simulink model "Model2"  (R2017a)
settings: Solver=ode23t  StartTime=0.0  StopTime=10.0  RelTol=1e-4
values from neighbouring files (symbols this model uses):
  param = evalin('base','param')    [getSaveInfo.m]    (also in loadBackUp.m)
(part 2 of 3)

== matlab function Model2/PodwojnyIntegrator/ObiektOdsprzegniety/Dynamika ==
  data: u input; zp output; q input; qp input; z input
function zp = fcn(u,q,qp,z)

c1=cos(q(6));
c3=cos(q(8));

s1=sin(q(6));
s3=sin(q(8));

invQ=[(0.679340444444444444E4+(-0.384000000000000000E3).*c1.^2+ ...
  0.407936888888888889E4.*c3+0.512000000000000000E3.*c1.*c3+( ...
  -0.170666666666666667E3).*c1.^2.*c3+(-0.162203728395061728E4).* ...
  c3.^2+0.113777777777777778E3.*c1.*c3.^2+0.125037037037037037E3.* ...
  c1.^2.*c3.^2+(-0.145391148148148148E4).*c3.^3+( ...
  -0.192000000000000000E3).*c1.*c3.^3+0.640000000000000000E2.* ...
  c1.^2.*c3.^3+(-0.347058518518518519E3).*c3.^4+( ...
  -0.426666666666666667E2).*c1.*c3.^4+0.711111111111111111E1.* ...
  c1.^2.*c3.^4+(-0.284444444444444444E2).*c3.^5+( ...
  -0.115200000000000000E4).*c1.*s1+0.768000000000000000E3.*c3.*s1+( ...
  -0.512000000000000000E3).*c1.*c3.*s1+0.170666666666666667E3.* ...
  c3.^2.*s1+0.375111111111111111E3.*c1.*c3.^2.*s1+( ...
  -0.288000000000000000E3).*c3.^3.*s1+0.192000000000000000E3.*c1.* ...
  c3.^3.*s1+(-0.640000000000000000E2).*c3.^4.*s1+ ...
  0.213333333333333333E2.*c1.*c3.^4.*s1+(-0.864000000000000000E3).* ...
  s1.^2+(-0.384000000000000000E3).*c3.*s1.^2+ ...
  0.281333333333333333E3.*c3.^2.*s1.^2+0.144000000000000000E3.* ...
  c3.^3.*s1.^2+0.160000000000000000E2.*c3.^4.*s1.^2+( ...
  -0.384000000000000000E3).*c1.^2.*s3.^2+(-0.192000000000000000E3).* ...
  c1.^2.*c3.*s3.^2+(-0.426666666666666667E2).*c1.^2.*c3.^2.*s3.^2+ ...
  0.512000000000000000E3.*c1.*s1.*s3.^2+0.256000000000000000E3.*c1.* ...
  c3.*s1.*s3.^2+0.568888888888888889E2.*c1.*c3.^2.*s1.*s3.^2+( ...
  -0.170666666666666667E3).*s1.^2.*s3.^2+(-0.853333333333333333E2).* ...
  c3.*s1.^2.*s3.^2+(-0.189629629629629630E2).*c3.^2.*s1.^2.*s3.^2).* ...
  (0.175621873777777778E7+0.E-37.*c1+(-0.236544000000000000E6).* ...
  c1.^2+0.129863203555555556E7.*c3+0.315392000000000000E6.*c1.*c3+( ...
  -0.105130666666666667E6).*c1.^2.*c3+(-0.358315944691358025E6).* ...
  c3.^2+0.700871111111111111E5.*c1.*c3.^2+0.770228148148148148E5.* ...
  c1.^2.*c3.^2+(-0.440262272592592593E6).*c3.^3+( ...
  -0.118272000000000000E6).*c1.*c3.^3+0.394240000000000000E5.* ...
  c1.^2.*c3.^3+(-0.112599780740740741E6).*c3.^4+( ...
  -0.262826666666666667E5).*c1.*c3.^4+0.438044444444444444E4.* ...
  c1.^2.*c3.^4+(-0.175217777777777778E5).*c3.^5+0.E-39.*c1.*c3.^5+ ...
  0.E-39.*c3.^6+0.E-36.*s1+0.E-37.*c1.*s1+0.E-37.*c3.*s1+0.E-37.* ...
  c1.*c3.*s1+0.E-37.*c3.^2.*s1+0.E-37.*c1.*c3.^2.*s1+0.E-37.*c3.^3.* ...
  s1+0.E-38.*c1.*c3.^3.*s1+0.E-38.*c3.^4.*s1+0.E-39.*c1.*c3.^4.*s1+ ...
  0.E-39.*c3.^5.*s1+(-0.384885600000000000E6).*s1.^2+( ...
  -0.263220266666666667E6).*c3.*s1.^2+0.843654037037037037E5.* ...
  c3.^2.*s1.^2+0.941564888888888889E5.*c3.^3.*s1.^2+ ...
  0.224875111111111111E5.*c3.^4.*s1.^2+0.170666666666666667E4.* ...
  c3.^5.*s1.^2+(-0.171060266666666667E6).*c1.^2.*s3.^2+ ...
  0.230400000000000000E5.*c1.^4.*s3.^2+(-0.126490133333333333E6).* ...
  c1.^2.*c3.*s3.^2+(-0.307200000000000000E5).*c1.^3.*c3.*s3.^2+ ...
  0.102400000000000000E5.*c1.^4.*c3.*s3.^2+(-0.292466962962962963E5) ...
  .*c1.^2.*c3.^2.*s3.^2+(-0.682666666666666667E4).*c1.^3.*c3.^2.* ...
  s3.^2+0.113777777777777778E4.*c1.^4.*c3.^2.*s3.^2+( ...
  -0.455111111111111111E4).*c1.^2.*c3.^3.*s3.^2+0.E-37.*c1.*s1.* ...
  s3.^2+0.E-37.*c1.*c3.*s1.*s3.^2+0.E-38.*c1.*c3.^2.*s1.*s3.^2+( ...
  -0.105130666666666667E6).*s1.^2.*s3.^2+0.460800000000000000E5.* ...
  c1.^2.*s1.^2.*s3.^2+(-0.525653333333333333E5).*c3.*s1.^2.*s3.^2+( ...
  -0.307200000000000000E5).*c1.*c3.*s1.^2.*s3.^2+ ...
  0.204800000000000000E5.*c1.^2.*c3.*s1.^2.*s3.^2+( ...
  -0.116811851851851852E5).*c3.^2.*s1.^2.*s3.^2+( ...
  -0.682666666666666667E4).*c1.*c3.^2.*s1.^2.*s3.^2+ ...
  0.227555555555555556E4.*c1.^2.*c3.^2.*s1.^2.*s3.^2+ ...
  0.230400000000000000E5.*s1.^4.*s3.^2+0.102400000000000000E5.*c3.* ...
  s1.^4.*s3.^2+0.113777777777777778E4.*c3.^2.*s1.^4.*s3.^2).^(-1),(( ...
  -0.109139555555555556E4)+(-0.384000000000000000E3).*c1.^2+ ...
  0.136968888888888889E3.*c3+0.512000000000000000E3.*c1.*c3+( ...
  -0.170666666666666667E3).*c1.^2.*c3+0.458673827160493827E3.*c3.^2+ ...
  0.113777777777777778E3.*c1.*c3.^2+0.125037037037037037E3.*c1.^2.* ...
  c3.^2+0.244885185185185185E2.*c3.^3+(-0.192000000000000000E3).* ...
  c1.*c3.^3+0.640000000000000000E2.*c1.^2.*c3.^3+( ...
  -0.185251851851851852E2).*c3.^4+(-0.426666666666666667E2).*c1.* ...
  c3.^4+0.711111111111111111E1.*c1.^2.*c3.^4+( ...
  -0.284444444444444444E2).*c3.^5+0.864000000000000000E3.*s1.^2+ ...
  0.384000000000000000E3.*c3.*s1.^2+(-0.281333333333333333E3).* ...
  c3.^2.*s1.^2+(-0.144000000000000000E3).*c3.^3.*s1.^2+( ...
  -0.160000000000000000E2).*c3.^4.*s1.^2+0.384000000000000000E3.* ...
  c1.^2.*s3.^2+0.192000000000000000E3.*c1.^2.*c3.*s3.^2+ ...
  0.426666666666666667E2.*c1.^2.*c3.^2.*s3.^2+( ...
  -0.170666666666666667E3).*s1.^2.*s3.^2+(-0.853333333333333333E2).* ...
  c3.*s1.^2.*s3.^2+(-0.189629629629629630E2).*c3.^2.*s1.^2.*s3.^2).* ...
  (0.175621873777777778E7+0.E-37.*c1+(-0.236544000000000000E6).* ...
  c1.^2+0.129863203555555556E7.*c3+0.315392000000000000E6.*c1.*c3+( ...
  -0.105130666666666667E6).*c1.^2.*c3+(-0.358315944691358025E6).* ...
  c3.^2+0.700871111111111111E5.*c1.*c3.^2+0.770228148148148148E5.* ...
  c1.^2.*c3.^2+(-0.440262272592592593E6).*c3.^3+( ...
  -0.118272000000000000E6).*c1.*c3.^3+0.394240000000000000E5.* ...
  c1.^2.*c3.^3+(-0.112599780740740741E6).*c3.^4+( ...
  -0.262826666666666667E5).*c1.*c3.^4+0.438044444444444444E4.* ...
  c1.^2.*c3.^4+(-0.175217777777777778E5).*c3.^5+0.E-39.*c1.*c3.^5+ ...
  0.E-39.*c3.^6+0.E-36.*s1+0.E-37.*c1.*s1+0.E-37.*c3.*s1+0.E-37.* ...
  c1.*c3.*s1+0.E-37.*c3.^2.*s1+0.E-37.*c1.*c3.^2.*s1+0.E-37.*c3.^3.* ...
  s1+0.E-38.*c1.*c3.^3.*s1+0.E-38.*c3.^4.*s1+0.E-39.*c1.*c3.^4.*s1+ ...
  0.E-39.*c3.^5.*s1+(-0.384885600000000000E6).*s1.^2+( ...
  -0.263220266666666667E6).*c3.*s1.^2+0.843654037037037037E5.* ...
  c3.^2.*s1.^2+0.941564888888888889E5.*c3.^3.*s1.^2+ ...
  0.224875111111111111E5.*c3.^4.*s1.^2+0.170666666666666667E4.* ...
  c3.^5.*s1.^2+(-0.171060266666666667E6).*c1.^2.*s3.^2+ ...
  0.230400000000000000E5.*c1.^4.*s3.^2+(-0.126490133333333333E6).* ...
  c1.^2.*c3.*s3.^2+(-0.307200000000000000E5).*c1.^3.*c3.*s3.^2+ ...
  0.102400000000000000E5.*c1.^4.*c3.*s3.^2+(-0.292466962962962963E5) ...
  .*c1.^2.*c3.^2.*s3.^2+(-0.682666666666666667E4).*c1.^3.*c3.^2.* ...
  s3.^2+0.113777777777777778E4.*c1.^4.*c3.^2.*s3.^2+( ...
  -0.455111111111111111E4).*c1.^2.*c3.^3.*s3.^2+0.E-37.*c1.*s1.* ...
  s3.^2+0.E-37.*c1.*c3.*s1.*s3.^2+0.E-38.*c1.*c3.^2.*s1.*s3.^2+( ...
  -0.105130666666666667E6).*s1.^2.*s3.^2+0.460800000000000000E5.* ...
  c1.^2.*s1.^2.*s3.^2+(-0.525653333333333333E5).*c3.*s1.^2.*s3.^2+( ...
  -0.307200000000000000E5).*c1.*c3.*s1.^2.*s3.^2+ ...
  0.204800000000000000E5.*c1.^2.*c3.*s1.^2.*s3.^2+( ...
  -0.116811851851851852E5).*c3.^2.*s1.^2.*s3.^2+( ...
  -0.682666666666666667E4).*c1.*c3.^2.*s1.^2.*s3.^2+ ...
  0.227555555555555556E4.*c1.^2.*c3.^2.*s1.^2.*s3.^2+ ...
  0.230400000000000000E5.*s1.^4.*s3.^2+0.102400000000000000E5.*c3.* ...
  s1.^4.*s3.^2+0.113777777777777778E4.*c3.^2.*s1.^4.*s3.^2).^(-1),(( ...
  -0.262826666666666667E5)+(-0.197120000000000000E5).*c1+( ...
  -0.438044444444444444E4).*c1.*c3+0.693570370370370370E4.*c3.^2+ ...
  0.739200000000000000E4.*c1.*c3.^2+0.164266666666666667E4.*c1.* ...
  c3.^3+0.109511111111111111E4.*c3.^4+0.213825333333333333E5.*s1+ ...
  0.384000000000000000E4.*c1.*s1+0.731167407407407407E4.*c3.*s1+ ...
  0.170666666666666667E4.*c1.*c3.*s1+(-0.744956111111111111E4).* ...
  c3.^2.*s1+(-0.125037037037037037E4).*c1.*c3.^2.*s1+( ...
  -0.274187777777777778E4).*c3.^3.*s1+(-0.640000000000000000E3).* ...
  c1.*c3.^3.*s1+(-0.213333333333333333E3).*c3.^4.*s1+( ...
  -0.711111111111111111E2).*c1.*c3.^4.*s1+0.576000000000000000E4.* ...
  s1.^2+0.256000000000000000E4.*c3.*s1.^2+(-0.187555555555555556E4) ...
  .*c3.^2.*s1.^2+(-0.960000000000000000E3).*c3.^3.*s1.^2+( ...
  -0.106666666666666667E3).*c3.^4.*s1.^2+0.256000000000000000E4.* ...
  c1.^2.*s3.^2+0.192000000000000000E4.*c1.^3.*s3.^2+ ...
  0.426666666666666667E3.*c1.^3.*c3.*s3.^2+0.284444444444444444E3.* ...
  c1.^2.*c3.^2.*s3.^2+(-0.170666666666666667E4).*c1.*s1.*s3.^2+( ...
  -0.128000000000000000E4).*c1.^2.*s1.*s3.^2+( ...
  -0.284444444444444444E3).*c1.^2.*c3.*s1.*s3.^2+( ...
  -0.189629629629629630E3).*c1.*c3.^2.*s1.*s3.^2+ ...
  0.192000000000000000E4.*c1.*s1.^2.*s3.^2+0.426666666666666667E3.* ...
  c1.*c3.*s1.^2.*s3.^2+(-0.128000000000000000E4).*s1.^3.*s3.^2+( ...
  -0.284444444444444444E3).*c3.*s1.^3.*s3.^2).*( ...
  0.175621873777777778E7+0.E-37.*c1+(-0.236544000000000000E6).* ...
  c1.^2+0.129863203555555556E7.*c3+0.315392000000000000E6.*c1.*c3+( ...
  -0.105130666666666667E6).*c1.^2.*c3+(-0.358315944691358025E6).* ...
  c3.^2+0.700871111111111111E5.*c1.*c3.^2+0.770228148148148148E5.* ...
  c1.^2.*c3.^2+(-0.440262272592592593E6).*c3.^3+( ...
  -0.118272000000000000E6).*c1.*c3.^3+0.394240000000000000E5.* ...
  c1.^2.*c3.^3+(-0.112599780740740741E6).*c3.^4+( ...
  -0.262826666666666667E5).*c1.*c3.^4+0.438044444444444444E4.* ...
  c1.^2.*c3.^4+(-0.175217777777777778E5).*c3.^5+0.E-39.*c1.*c3.^5+ ...
  0.E-39.*c3.^6+0.E-36.*s1+0.E-37.*c1.*s1+0.E-37.*c3.*s1+0.E-37.* ...
  c1.*c3.*s1+0.E-37.*c3.^2.*s1+0.E-37.*c1.*c3.^2.*s1+0.E-37.*c3.^3.* ...
  s1+0.E-38.*c1.*c3.^3.*s1+0.E-38.*c3.^4.*s1+0.E-39.*c1.*c3.^4.*s1+ ...
  0.E-39.*c3.^5.*s1+(-0.384885600000000000E6).*s1.^2+( ...
  -0.263220266666666667E6).*c3.*s1.^2+0.843654037037037037E5.* ...
  c3.^2.*s1.^2+0.941564888888888889E5.*c3.^3.*s1.^2+ ...
  0.224875111111111111E5.*c3.^4.*s1.^2+0.170666666666666667E4.* ...
  c3.^5.*s1.^2+(-0.171060266666666667E6).*c1.^2.*s3.^2+ ...
  0.230400000000000000E5.*c1.^4.*s3.^2+(-0.126490133333333333E6).* ...
  c1.^2.*c3.*s3.^2+(-0.307200000000000000E5).*c1.^3.*c3.*s3.^2+ ...
  0.102400000000000000E5.*c1.^4.*c3.*s3.^2+(-0.292466962962962963E5) ...
  .*c1.^2.*c3.^2.*s3.^2+(-0.682666666666666667E4).*c1.^3.*c3.^2.* ...
  s3.^2+0.113777777777777778E4.*c1.^4.*c3.^2.*s3.^2+( ...
  -0.455111111111111111E4).*c1.^2.*c3.^3.*s3.^2+0.E-37.*c1.*s1.* ...
  s3.^2+0.E-37.*c1.*c3.*s1.*s3.^2+0.E-38.*c1.*c3.^2.*s1.*s3.^2+( ...
  -0.105130666666666667E6).*s1.^2.*s3.^2+0.460800000000000000E5.* ...
  c1.^2.*s1.^2.*s3.^2+(-0.525653333333333333E5).*c3.*s1.^2.*s3.^2+( ...
  -0.307200000000000000E5).*c1.*c3.*s1.^2.*s3.^2+ ...
  0.204800000000000000E5.*c1.^2.*c3.*s1.^2.*s3.^2+( ...
  -0.116811851851851852E5).*c3.^2.*s1.^2.*s3.^2+( ...
  -0.682666666666666667E4).*c1.*c3.^2.*s1.^2.*s3.^2+ ...
  0.227555555555555556E4.*c1.^2.*c3.^2.*s1.^2.*s3.^2+ ...
  0.230400000000000000E5.*s1.^4.*s3.^2+0.102400000000000000E5.*c3.* ...
  s1.^4.*s3.^2+0.113777777777777778E4.*c3.^2.*s1.^4.*s3.^2).^(-1),(( ...
  -0.213825333333333333E4).*c1.*c3.*s3+0.288000000000000000E3.* ...
  c1.^3.*c3.*s3+(-0.158112666666666667E4).*c1.*c3.^2.*s3+( ...
  -0.384000000000000000E3).*c1.^2.*c3.^2.*s3+ ...
  0.128000000000000000E3.*c1.^3.*c3.^2.*s3+(-0.365583703703703704E3) ...
  .*c1.*c3.^3.*s3+(-0.853333333333333333E2).*c1.^2.*c3.^3.*s3+ ...
  0.142222222222222222E2.*c1.^3.*c3.^3.*s3+(-0.568888888888888889E2) ...
  .*c1.*c3.^4.*s3+(-0.197120000000000000E4).*c3.*s1.*s3+ ...
  0.432000000000000000E3.*c1.^2.*c3.*s1.*s3+( ...
  -0.985600000000000000E3).*c3.^2.*s1.*s3+(-0.288000000000000000E3) ...
  .*c1.*c3.^2.*s1.*s3+0.192000000000000000E3.*c1.^2.*c3.^2.*s1.*s3+( ...
  -0.219022222222222222E3).*c3.^3.*s1.*s3+(-0.640000000000000000E2) ...
  .*c1.*c3.^3.*s1.*s3+0.213333333333333333E2.*c1.^2.*c3.^3.*s1.*s3+ ...
  0.288000000000000000E3.*c1.*c3.*s1.^2.*s3+( ...
  -0.192000000000000000E3).*c3.^2.*s1.^2.*s3+ ...
  0.128000000000000000E3.*c1.*c3.^2.*s1.^2.*s3+( ...
  -0.426666666666666667E2).*c3.^3.*s1.^2.*s3+ ...
  0.142222222222222222E2.*c1.*c3.^3.*s1.^2.*s3+ ...
  0.432000000000000000E3.*c3.*s1.^3.*s3+0.192000000000000000E3.* ...
  c3.^2.*s1.^3.*s3+0.213333333333333333E2.*c3.^3.*s1.^3.*s3).*( ...
  0.175621873777777778E7+0.E-37.*c1+(-0.236544000000000000E6).* ...
  c1.^2+0.129863203555555556E7.*c3+0.315392000000000000E6.*c1.*c3+( ...
  -0.105130666666666667E6).*c1.^2.*c3+(-0.358315944691358025E6).* ...
  c3.^2+0.700871111111111111E5.*c1.*c3.^2+0.770228148148148148E5.* ...
  c1.^2.*c3.^2+(-0.440262272592592593E6).*c3.^3+( ...
  -0.118272000000000000E6).*c1.*c3.^3+0.394240000000000000E5.* ...
  c1.^2.*c3.^3+(-0.112599780740740741E6).*c3.^4+( ...
  -0.262826666666666667E5).*c1.*c3.^4+0.438044444444444444E4.* ...
  c1.^2.*c3.^4+(-0.175217777777777778E5).*c3.^5+0.E-39.*c1.*c3.^5+ ...
  0.E-39.*c3.^6+0.E-36.*s1+0.E-37.*c1.*s1+0.E-37.*c3.*s1+0.E-37.* ...
  c1.*c3.*s1+0.E-37.*c3.^2.*s1+0.E-37.*c1.*c3.^2.*s1+0.E-37.*c3.^3.* ...
  s1+0.E-38.*c1.*c3.^3.*s1+0.E-38.*c3.^4.*s1+0.E-39.*c1.*c3.^4.*s1+ ...
  0.E-39.*c3.^5.*s1+(-0.384885600000000000E6).*s1.^2+( ...
  -0.263220266666666667E6).*c3.*s1.^2+0.843654037037037037E5.* ...
  c3.^2.*s1.^2+0.941564888888888889E5.*c3.^3.*s1.^2+ ...
  0.224875111111111111E5.*c3.^4.*s1.^2+0.170666666666666667E4.* ...
  c3.^5.*s1.^2+(-0.171060266666666667E6).*c1.^2.*s3.^2+ ...
  0.230400000000000000E5.*c1.^4.*s3.^2+(-0.126490133333333333E6).* ...
  c1.^2.*c3.*s3.^2+(-0.307200000000000000E5).*c1.^3.*c3.*s3.^2+ ...
  0.102400000000000000E5.*c1.^4.*c3.*s3.^2+(-0.292466962962962963E5) ...
  .*c1.^2.*c3.^2.*s3.^2+(-0.682666666666666667E4).*c1.^3.*c3.^2.* ...
  s3.^2+0.113777777777777778E4.*c1.^4.*c3.^2.*s3.^2+( ...
  -0.455111111111111111E4).*c1.^2.*c3.^3.*s3.^2+0.E-37.*c1.*s1.* ...
  s3.^2+0.E-37.*c1.*c3.*s1.*s3.^2+0.E-38.*c1.*c3.^2.*s1.*s3.^2+( ...
  -0.105130666666666667E6).*s1.^2.*s3.^2+0.460800000000000000E5.* ...
  c1.^2.*s1.^2.*s3.^2+(-0.525653333333333333E5).*c3.*s1.^2.*s3.^2+( ...
  -0.307200000000000000E5).*c1.*c3.*s1.^2.*s3.^2+ ...
  0.204800000000000000E5.*c1.^2.*c3.*s1.^2.*s3.^2+( ...
  -0.116811851851851852E5).*c3.^2.*s1.^2.*s3.^2+( ...
  -0.682666666666666667E4).*c1.*c3.^2.*s1.^2.*s3.^2+ ...
  0.227555555555555556E4.*c1.^2.*c3.^2.*s1.^2.*s3.^2+ ...
  0.230400000000000000E5.*s1.^4.*s3.^2+0.102400000000000000E5.*c3.* ...
  s1.^4.*s3.^2+0.113777777777777778E4.*c3.^2.*s1.^4.*s3.^2).^(-1),( ...
  0.427650666666666667E5.*c1.*s3+(-0.576000000000000000E4).*c1.^3.* ...
  s3+0.316225333333333333E5.*c1.*c3.*s3+0.768000000000000000E4.* ...
  c1.^2.*c3.*s3+(-0.256000000000000000E4).*c1.^3.*c3.*s3+ ...
  0.731167407407407407E4.*c1.*c3.^2.*s3+0.170666666666666667E4.* ...
  c1.^2.*c3.^2.*s3+(-0.284444444444444444E3).*c1.^3.*c3.^2.*s3+ ...
  0.113777777777777778E4.*c1.*c3.^3.*s3+0.394240000000000000E5.*s1.* ...
  s3+(-0.864000000000000000E4).*c1.^2.*s1.*s3+ ...
  0.197120000000000000E5.*c3.*s1.*s3+0.576000000000000000E4.*c1.* ...
  c3.*s1.*s3+(-0.384000000000000000E4).*c1.^2.*c3.*s1.*s3+ ...
  0.438044444444444444E4.*c3.^2.*s1.*s3+0.128000000000000000E4.*c1.* ...
  c3.^2.*s1.*s3+(-0.426666666666666667E3).*c1.^2.*c3.^2.*s1.*s3+( ...
  -0.576000000000000000E4).*c1.*s1.^2.*s3+0.384000000000000000E4.* ...
  c3.*s1.^2.*s3+(-0.256000000000000000E4).*c1.*c3.*s1.^2.*s3+ ...
  0.853333333333333333E3.*c3.^2.*s1.^2.*s3+(-0.284444444444444444E3) ...
  .*c1.*c3.^2.*s1.^2.*s3+(-0.864000000000000000E4).*s1.^3.*s3+( ...
  -0.384000000000000000E4).*c3.*s1.^3.*s3+(-0.426666666666666667E3) ...
  .*c3.^2.*s1.^3.*s3).*(0.175621873777777778E7+0.E-37.*c1+( ...
  -0.236544000000000000E6).*c1.^2+0.129863203555555556E7.*c3+ ...
  0.315392000000000000E6.*c1.*c3+(-0.105130666666666667E6).*c1.^2.* ...
  c3+(-0.358315944691358025E6).*c3.^2+0.700871111111111111E5.*c1.* ...
  c3.^2+0.770228148148148148E5.*c1.^2.*c3.^2+( ...
  -0.440262272592592593E6).*c3.^3+(-0.118272000000000000E6).*c1.* ...
  c3.^3+0.394240000000000000E5.*c1.^2.*c3.^3+( ...
  -0.112599780740740741E6).*c3.^4+(-0.262826666666666667E5).*c1.* ...
  c3.^4+0.438044444444444444E4.*c1.^2.*c3.^4+( ...
  -0.175217777777777778E5).*c3.^5+0.E-39.*c1.*c3.^5+0.E-39.*c3.^6+ ...
  0.E-36.*s1+0.E-37.*c1.*s1+0.E-37.*c3.*s1+0.E-37.*c1.*c3.*s1+ ...
  0.E-37.*c3.^2.*s1+0.E-37.*c1.*c3.^2.*s1+0.E-37.*c3.^3.*s1+0.E-38.* ...
  c1.*c3.^3.*s1+0.E-38.*c3.^4.*s1+0.E-39.*c1.*c3.^4.*s1+0.E-39.* ...
  c3.^5.*s1+(-0.384885600000000000E6).*s1.^2+( ...
  -0.263220266666666667E6).*c3.*s1.^2+0.843654037037037037E5.* ...
  c3.^2.*s1.^2+0.941564888888888889E5.*c3.^3.*s1.^2+ ...
  0.224875111111111111E5.*c3.^4.*s1.^2+0.170666666666666667E4.* ...
  c3.^5.*s1.^2+(-0.171060266666666667E6).*c1.^2.*s3.^2+ ...
  0.230400000000000000E5.*c1.^4.*s3.^2+(-0.126490133333333333E6).* ...
  c1.^2.*c3.*s3.^2+(-0.307200000000000000E5).*c1.^3.*c3.*s3.^2+ ...
  0.102400000000000000E5.*c1.^4.*c3.*s3.^2+(-0.292466962962962963E5) ...
  .*c1.^2.*c3.^2.*s3.^2+(-0.682666666666666667E4).*c1.^3.*c3.^2.* ...
  s3.^2+0.113777777777777778E4.*c1.^4.*c3.^2.*s3.^2+( ...
  -0.455111111111111111E4).*c1.^2.*c3.^3.*s3.^2+0.E-37.*c1.*s1.* ...
  s3.^2+0.E-37.*c1.*c3.*s1.*s3.^2+0.E-38.*c1.*c3.^2.*s1.*s3.^2+( ...
  -0.105130666666666667E6).*s1.^2.*s3.^2+0.460800000000000000E5.* ...
  c1.^2.*s1.^2.*s3.^2+(-0.525653333333333333E5).*c3.*s1.^2.*s3.^2+( ...
  -0.307200000000000000E5).*c1.*c3.*s1.^2.*s3.^2+ ...
  0.204800000000000000E5.*c1.^2.*c3.*s1.^2.*s3.^2+( ...
  -0.116811851851851852E5).*c3.^2.*s1.^2.*s3.^2+( ...
  -0.682666666666666667E4).*c1.*c3.^2.*s1.^2.*s3.^2+ ...
  0.227555555555555556E4.*c1.^2.*c3.^2.*s1.^2.*s3.^2+ ...
  0.230400000000000000E5.*s1.^4.*s3.^2+0.102400000000000000E5.*c3.* ...
  s1.^4.*s3.^2+0.113777777777777778E4.*c3.^2.*s1.^4.*s3.^2).^(-1);(( ...
  -0.109139555555555556E4)+(-0.384000000000000000E3).*c1.^2+ ...
  0.136968888888888889E3.*c3+0.512000000000000000E3.*c1.*c3+( ...
  -0.170666666666666667E3).*c1.^2.*c3+0.458673827160493827E3.*c3.^2+ ...
  0.113777777777777778E3.*c1.*c3.^2+0.125037037037037037E3.*c1.^2.* ...
  c3.^2+0.244885185185185185E2.*c3.^3+(-0.192000000000000000E3).* ...
  c1.*c3.^3+0.640000000000000000E2.*c1.^2.*c3.^3+( ...
  -0.185251851851851852E2).*c3.^4+(-0.426666666666666667E2).*c1.* ...
  c3.^4+0.711111111111111111E1.*c1.^2.*c3.^4+( ...
  -0.284444444444444444E2).*c3.^5+0.864000000000000000E3.*s1.^2+ ...
  0.384000000000000000E3.*c3.*s1.^2+(-0.281333333333333333E3).* ...
  c3.^2.*s1.^2+(-0.144000000000000000E3).*c3.^3.*s1.^2+( ...
  -0.160000000000000000E2).*c3.^4.*s1.^2+0.384000000000000000E3.* ...
  c1.^2.*s3.^2+0.192000000000000000E3.*c1.^2.*c3.*s3.^2+ ...
  0.426666666666666667E2.*c1.^2.*c3.^2.*s3.^2+( ...
  -0.170666666666666667E3).*s1.^2.*s3.^2+(-0.853333333333333333E2).* ...
  c3.*s1.^2.*s3.^2+(-0.189629629629629630E2).*c3.^2.*s1.^2.*s3.^2).* ...
  (0.175621873777777778E7+0.E-37.*c1+(-0.236544000000000000E6).* ...
  c1.^2+0.129863203555555556E7.*c3+0.315392000000000000E6.*c1.*c3+( ...
  -0.105130666666666667E6).*c1.^2.*c3+(-0.358315944691358025E6).* ...
  c3.^2+0.700871111111111111E5.*c1.*c3.^2+0.770228148148148148E5.* ...
  c1.^2.*c3.^2+(-0.440262272592592593E6).*c3.^3+( ...
  -0.118272000000000000E6).*c1.*c3.^3+0.394240000000000000E5.* ...
  c1.^2.*c3.^3+(-0.112599780740740741E6).*c3.^4+( ...
  -0.262826666666666667E5).*c1.*c3.^4+0.438044444444444444E4.* ...
  c1.^2.*c3.^4+(-0.175217777777777778E5).*c3.^5+0.E-39.*c1.*c3.^5+ ...
  0.E-39.*c3.^6+0.E-36.*s1+0.E-37.*c1.*s1+0.E-37.*c3.*s1+0.E-37.* ...
  c1.*c3.*s1+0.E-37.*c3.^2.*s1+0.E-37.*c1.*c3.^2.*s1+0.E-37.*c3.^3.* ...
  s1+0.E-38.*c1.*c3.^3.*s1+0.E-38.*c3.^4.*s1+0.E-39.*c1.*c3.^4.*s1+ ...
  0.E-39.*c3.^5.*s1+(-0.384885600000000000E6).*s1.^2+( ...
  -0.263220266666666667E6).*c3.*s1.^2+0.843654037037037037E5.* ...
  c3.^2.*s1.^2+0.941564888888888889E5.*c3.^3.*s1.^2+ ...
  0.224875111111111111E5.*c3.^4.*s1.^2+0.170666666666666667E4.* ...
  c3.^5.*s1.^2+(-0.171060266666666667E6).*c1.^2.*s3.^2+ ...
  0.230400000000000000E5.*c1.^4.*s3.^2+(-0.126490133333333333E6).* ...
  c1.^2.*c3.*s3.^2+(-0.307200000000000000E5).*c1.^3.*c3.*s3.^2+ ...
  0.102400000000000000E5.*c1.^4.*c3.*s3.^2+(-0.292466962962962963E5) ...
  .*c1.^2.*c3.^2.*s3.^2+(-0.682666666666666667E4).*c1.^3.*c3.^2.* ...
  s3.^2+0.113777777777777778E4.*c1.^4.*c3.^2.*s3.^2+( ...
  -0.455111111111111111E4).*c1.^2.*c3.^3.*s3.^2+0.E-37.*c1.*s1.* ...
  s3.^2+0.E-37.*c1.*c3.*s1.*s3.^2+0.E-38.*c1.*c3.^2.*s1.*s3.^2+( ...
  -0.105130666666666667E6).*s1.^2.*s3.^2+0.460800000000000000E5.* ...
  c1.^2.*s1.^2.*s3.^2+(-0.525653333333333333E5).*c3.*s1.^2.*s3.^2+( ...
  -0.307200000000000000E5).*c1.*c3.*s1.^2.*s3.^2+ ...
  0.204800000000000000E5.*c1.^2.*c3.*s1.^2.*s3.^2+( ...
  -0.116811851851851852E5).*c3.^2.*s1.^2.*s3.^2+( ...
  -0.682666666666666667E4).*c1.*c3.^2.*s1.^2.*s3.^2+ ...
  0.227555555555555556E4.*c1.^2.*c3.^2.*s1.^2.*s3.^2+ ...
  0.230400000000000000E5.*s1.^4.*s3.^2+0.102400000000000000E5.*c3.* ...
  s1.^4.*s3.^2+0.113777777777777778E4.*c3.^2.*s1.^4.*s3.^2).^(-1),( ...
  0.679340444444444444E4+(-0.384000000000000000E3).*c1.^2+ ...
  0.407936888888888889E4.*c3+0.512000000000000000E3.*c1.*c3+( ...
  -0.170666666666666667E3).*c1.^2.*c3+(-0.162203728395061728E4).* ...
  c3.^2+0.113777777777777778E3.*c1.*c3.^2+0.125037037037037037E3.* ...
  c1.^2.*c3.^2+(-0.145391148148148148E4).*c3.^3+( ...
  -0.192000000000000000E3).*c1.*c3.^3+0.640000000000000000E2.* ...
  c1.^2.*c3.^3+(-0.347058518518518519E3).*c3.^4+( ...
  -0.426666666666666667E2).*c1.*c3.^4+0.711111111111111111E1.* ...
  c1.^2.*c3.^4+(-0.284444444444444444E2).*c3.^5+ ...
  0.115200000000000000E4.*c1.*s1+(-0.768000000000000000E3).*c3.*s1+ ...
  0.512000000000000000E3.*c1.*c3.*s1+(-0.170666666666666667E3).* ...
  c3.^2.*s1+(-0.375111111111111111E3).*c1.*c3.^2.*s1+ ...
  0.288000000000000000E3.*c3.^3.*s1+(-0.192000000000000000E3).*c1.* ...
  c3.^3.*s1+0.640000000000000000E2.*c3.^4.*s1+( ...
  -0.213333333333333333E2).*c1.*c3.^4.*s1+(-0.864000000000000000E3) ...
  .*s1.^2+(-0.384000000000000000E3).*c3.*s1.^2+ ...
  0.281333333333333333E3.*c3.^2.*s1.^2+0.144000000000000000E3.* ...
  c3.^3.*s1.^2+0.160000000000000000E2.*c3.^4.*s1.^2+( ...
  -0.384000000000000000E3).*c1.^2.*s3.^2+(-0.192000000000000000E3).* ...
  c1.^2.*c3.*s3.^2+(-0.426666666666666667E2).*c1.^2.*c3.^2.*s3.^2+( ...
  -0.512000000000000000E3).*c1.*s1.*s3.^2+(-0.256000000000000000E3) ...
  .*c1.*c3.*s1.*s3.^2+(-0.568888888888888889E2).*c1.*c3.^2.*s1.* ...
  s3.^2+(-0.170666666666666667E3).*s1.^2.*s3.^2+( ...
  -0.853333333333333333E2).*c3.*s1.^2.*s3.^2+( ...
  -0.189629629629629630E2).*c3.^2.*s1.^2.*s3.^2).*( ...
  0.175621873777777778E7+0.E-37.*c1+(-0.236544000000000000E6).* ...
  c1.^2+0.129863203555555556E7.*c3+0.315392000000000000E6.*c1.*c3+( ...
  -0.105130666666666667E6).*c1.^2.*c3+(-0.358315944691358025E6).* ...
  c3.^2+0.700871111111111111E5.*c1.*c3.^2+0.770228148148148148E5.* ...
  c1.^2.*c3.^2+(-0.440262272592592593E6).*c3.^3+( ...
  -0.118272000000000000E6).*c1.*c3.^3+0.394240000000000000E5.* ...
  c1.^2.*c3.^3+(-0.112599780740740741E6).*c3.^4+( ...
  -0.262826666666666667E5).*c1.*c3.^4+0.438044444444444444E4.* ...
  c1.^2.*c3.^4+(-0.175217777777777778E5).*c3.^5+0.E-39.*c1.*c3.^5+ ...
  0.E-39.*c3.^6+0.E-36.*s1+0.E-37.*c1.*s1+0.E-37.*c3.*s1+0.E-37.* ...
  c1.*c3.*s1+0.E-37.*c3.^2.*s1+0.E-37.*c1.*c3.^2.*s1+0.E-37.*c3.^3.* ...
  s1+0.E-38.*c1.*c3.^3.*s1+0.E-38.*c3.^4.*s1+0.E-39.*c1.*c3.^4.*s1+ ...
  0.E-39.*c3.^5.*s1+(-0.384885600000000000E6).*s1.^2+( ...
  -0.263220266666666667E6).*c3.*s1.^2+0.843654037037037037E5.* ...
  c3.^2.*s1.^2+0.941564888888888889E5.*c3.^3.*s1.^2+ ...
  0.224875111111111111E5.*c3.^4.*s1.^2+0.170666666666666667E4.* ...
  c3.^5.*s1.^2+(-0.171060266666666667E6).*c1.^2.*s3.^2+ ...
  0.230400000000000000E5.*c1.^4.*s3.^2+(-0.126490133333333333E6).* ...
  c1.^2.*c3.*s3.^2+(-0.307200000000000000E5).*c1.^3.*c3.*s3.^2+ ...
  0.102400000000000000E5.*c1.^4.*c3.*s3.^2+(-0.292466962962962963E5) ...
  .*c1.^2.*c3.^2.*s3.^2+(-0.682666666666666667E4).*c1.^3.*c3.^2.* ...
  s3.^2+0.113777777777777778E4.*c1.^4.*c3.^2.*s3.^2+( ...
  -0.455111111111111111E4).*c1.^2.*c3.^3.*s3.^2+0.E-37.*c1.*s1.* ...
  s3.^2+0.E-37.*c1.*c3.*s1.*s3.^2+0.E-38.*c1.*c3.^2.*s1.*s3.^2+( ...
  -0.105130666666666667E6).*s1.^2.*s3.^2+0.460800000000000000E5.* ...
  c1.^2.*s1.^2.*s3.^2+(-0.525653333333333333E5).*c3.*s1.^2.*s3.^2+( ...
  -0.307200000000000000E5).*c1.*c3.*s1.^2.*s3.^2+ ...
  0.204800000000000000E5.*c1.^2.*c3.*s1.^2.*s3.^2+( ...
  -0.116811851851851852E5).*c3.^2.*s1.^2.*s3.^2+( ...
  -0.682666666666666667E4).*c1.*c3.^2.*s1.^2.*s3.^2+ ...
  0.227555555555555556E4.*c1.^2.*c3.^2.*s1.^2.*s3.^2+ ...
  0.230400000000000000E5.*s1.^4.*s3.^2+0.102400000000000000E5.*c3.* ...
  s1.^4.*s3.^2+0.113777777777777778E4.*c3.^2.*s1.^4.*s3.^2).^(-1),( ...
  0.262826666666666667E5+0.197120000000000000E5.*c1+ ...
  0.438044444444444444E4.*c1.*c3+(-0.693570370370370370E4).*c3.^2+( ...
  -0.739200000000000000E4).*c1.*c3.^2+(-0.164266666666666667E4).* ...
  c1.*c3.^3+(-0.109511111111111111E4).*c3.^4+ ...
  0.213825333333333333E5.*s1+0.384000000000000000E4.*c1.*s1+ ...
  0.731167407407407407E4.*c3.*s1+0.170666666666666667E4.*c1.*c3.*s1+ ...
  (-0.744956111111111111E4).*c3.^2.*s1+(-0.125037037037037037E4).* ...
  c1.*c3.^2.*s1+(-0.274187777777777778E4).*c3.^3.*s1+( ...
  -0.640000000000000000E3).*c1.*c3.^3.*s1+(-0.213333333333333333E3) ...
  .*c3.^4.*s1+(-0.711111111111111111E2).*c1.*c3.^4.*s1+( ...
  -0.576000000000000000E4).*s1.^2+(-0.256000000000000000E4).*c3.* ...
  s1.^2+0.187555555555555556E4.*c3.^2.*s1.^2+ ...
  0.960000000000000000E3.*c3.^3.*s1.^2+0.106666666666666667E3.* ...
  c3.^4.*s1.^2+(-0.256000000000000000E4).*c1.^2.*s3.^2+( ...
  -0.192000000000000000E4).*c1.^3.*s3.^2+(-0.426666666666666667E3).* ...
  c1.^3.*c3.*s3.^2+(-0.284444444444444444E3).*c1.^2.*c3.^2.*s3.^2+( ...
  -0.170666666666666667E4).*c1.*s1.*s3.^2+(-0.128000000000000000E4) ...
  .*c1.^2.*s1.*s3.^2+(-0.284444444444444444E3).*c1.^2.*c3.*s1.* ...
  s3.^2+(-0.189629629629629630E3).*c1.*c3.^2.*s1.*s3.^2+( ...
  -0.192000000000000000E4).*c1.*s1.^2.*s3.^2+( ...
  -0.426666666666666667E3).*c1.*c3.*s1.^2.*s3.^2+( ...
  -0.128000000000000000E4).*s1.^3.*s3.^2+(-0.284444444444444444E3).* ...
  c3.*s1.^3.*s3.^2).*(0.175621873777777778E7+0.E-37.*c1+( ...
  -0.236544000000000000E6).*c1.^2+0.129863203555555556E7.*c3+ ...
  0.315392000000000000E6.*c1.*c3+(-0.105130666666666667E6).*c1.^2.* ...
  c3+(-0.358315944691358025E6).*c3.^2+0.700871111111111111E5.*c1.* ...
  c3.^2+0.770228148148148148E5.*c1.^2.*c3.^2+( ...
  -0.440262272592592593E6).*c3.^3+(-0.118272000000000000E6).*c1.* ...
  c3.^3+0.394240000000000000E5.*c1.^2.*c3.^3+( ...
  -0.112599780740740741E6).*c3.^4+(-0.262826666666666667E5).*c1.* ...
  c3.^4+0.438044444444444444E4.*c1.^2.*c3.^4+( ...
  -0.175217777777777778E5).*c3.^5+0.E-39.*c1.*c3.^5+0.E-39.*c3.^6+ ...
  0.E-36.*s1+0.E-37.*c1.*s1+0.E-37.*c3.*s1+0.E-37.*c1.*c3.*s1+ ...
  0.E-37.*c3.^2.*s1+0.E-37.*c1.*c3.^2.*s1+0.E-37.*c3.^3.*s1+0.E-38.* ...
  c1.*c3.^3.*s1+0.E-38.*c3.^4.*s1+0.E-39.*c1.*c3.^4.*s1+0.E-39.* ...
  c3.^5.*s1+(-0.384885600000000000E6).*s1.^2+( ...
  -0.263220266666666667E6).*c3.*s1.^2+0.843654037037037037E5.* ...
  c3.^2.*s1.^2+0.941564888888888889E5.*c3.^3.*s1.^2+ ...
  0.224875111111111111E5.*c3.^4.*s1.^2+0.170666666666666667E4.* ...
  c3.^5.*s1.^2+(-0.171060266666666667E6).*c1.^2.*s3.^2+ ...
  0.230400000000000000E5.*c1.^4.*s3.^2+(-0.126490133333333333E6).* ...
  c1.^2.*c3.*s3.^2+(-0.307200000000000000E5).*c1.^3.*c3.*s3.^2+ ...
  0.102400000000000000E5.*c1.^4.*c3.*s3.^2+(-0.292466962962962963E5) ...
  .*c1.^2.*c3.^2.*s3.^2+(-0.682666666666666667E4).*c1.^3.*c3.^2.* ...
  s3.^2+0.113777777777777778E4.*c1.^4.*c3.^2.*s3.^2+( ...
  -0.455111111111111111E4).*c1.^2.*c3.^3.*s3.^2+0.E-37.*c1.*s1.* ...
  s3.^2+0.E-37.*c1.*c3.*s1.*s3.^2+0.E-38.*c1.*c3.^2.*s1.*s3.^2+( ...
  -0.105130666666666667E6).*s1.^2.*s3.^2+0.460800000000000000E5.* ...
  c1.^2.*s1.^2.*s3.^2+(-0.525653333333333333E5).*c3.*s1.^2.*s3.^2+( ...
  -0.307200000000000000E5).*c1.*c3.*s1.^2.*s3.^2+ ...
  0.204800000000000000E5.*c1.^2.*c3.*s1.^2.*s3.^2+( ...
  -0.116811851851851852E5).*c3.^2.*s1.^2.*s3.^2+( ...
  -0.682666666666666667E4).*c1.*c3.^2.*s1.^2.*s3.^2+ ...
  0.227555555555555556E4.*c1.^2.*c3.^2.*s1.^2.*s3.^2+ ...
  0.230400000000000000E5.*s1.^4.*s3.^2+0.102400000000000000E5.*c3.* ...
  s1.^4.*s3.^2+0.113777777777777778E4.*c3.^2.*s1.^4.*s3.^2).^(-1),(( ...
  -0.213825333333333333E4).*c1.*c3.*s3+0.288000000000000000E3.* ...
  c1.^3.*c3.*s3+(-0.158112666666666667E4).*c1.*c3.^2.*s3+( ...
  -0.384000000000000000E3).*c1.^2.*c3.^2.*s3+ ...
  0.128000000000000000E3.*c1.^3.*c3.^2.*s3+(-0.365583703703703704E3) ...
  .*c1.*c3.^3.*s3+(-0.853333333333333333E2).*c1.^2.*c3.^3.*s3+ ...
  0.142222222222222222E2.*c1.^3.*c3.^3.*s3+(-0.568888888888888889E2) ...
  .*c1.*c3.^4.*s3+0.197120000000000000E4.*c3.*s1.*s3+( ...
  -0.432000000000000000E3).*c1.^2.*c3.*s1.*s3+ ...
  0.985600000000000000E3.*c3.^2.*s1.*s3+0.288000000000000000E3.*c1.* ...
  c3.^2.*s1.*s3+(-0.192000000000000000E3).*c1.^2.*c3.^2.*s1.*s3+ ...
  0.219022222222222222E3.*c3.^3.*s1.*s3+0.640000000000000000E2.*c1.* ...
  c3.^3.*s1.*s3+(-0.213333333333333333E2).*c1.^2.*c3.^3.*s1.*s3+ ...
  0.288000000000000000E3.*c1.*c3.*s1.^2.*s3+( ...
  -0.192000000000000000E3).*c3.^2.*s1.^2.*s3+ ...
  0.128000000000000000E3.*c1.*c3.^2.*s1.^2.*s3+( ...
  -0.426666666666666667E2).*c3.^3.*s1.^2.*s3+ ...
  0.142222222222222222E2.*c1.*c3.^3.*s1.^2.*s3+( ...
  -0.432000000000000000E3).*c3.*s1.^3.*s3+(-0.192000000000000000E3) ...
  .*c3.^2.*s1.^3.*s3+(-0.213333333333333333E2).*c3.^3.*s1.^3.*s3).*( ...
  0.175621873777777778E7+0.E-37.*c1+(-0.236544000000000000E6).* ...
  c1.^2+0.129863203555555556E7.*c3+0.315392000000000000E6.*c1.*c3+( ...
  -0.105130666666666667E6).*c1.^2.*c3+(-0.358315944691358025E6).* ...
  c3.^2+0.700871111111111111E5.*c1.*c3.^2+0.770228148148148148E5.* ...
  c1.^2.*c3.^2+(-0.440262272592592593E6).*c3.^3+( ...
  -0.118272000000000000E6).*c1.*c3.^3+0.394240000000000000E5.* ...
  c1.^2.*c3.^3+(-0.112599780740740741E6).*c3.^4+( ...
  -0.262826666666666667E5).*c1.*c3.^4+0.438044444444444444E4.* ...
  c1.^2.*c3.^4+(-0.175217777777777778E5).*c3.^5+0.E-39.*c1.*c3.^5+ ...
  0.E-39.*c3.^6+0.E-36.*s1+0.E-37.*c1.*s1+0.E-37.*c3.*s1+0.E-37.* ...
  c1.*c3.*s1+0.E-37.*c3.^2.*s1+0.E-37.*c1.*c3.^2.*s1+0.E-37.*c3.^3.* ...
  s1+0.E-38.*c1.*c3.^3.*s1+0.E-38.*c3.^4.*s1+0.E-39.*c1.*c3.^4.*s1+ ...
  0.E-39.*c3.^5.*s1+(-0.384885600000000000E6).*s1.^2+( ...
  -0.263220266666666667E6).*c3.*s1.^2+0.843654037037037037E5.* ...
  c3.^2.*s1.^2+0.941564888888888889E5.*c3.^3.*s1.^2+ ...
  0.224875111111111111E5.*c3.^4.*s1.^2+0.170666666666666667E4.* ...
  c3.^5.*s1.^2+(-0.171060266666666667E6).*c1.^2.*s3.^2+ ...
  0.230400000000000000E5.*c1.^4.*s3.^2+(-0.126490133333333333E6).* ...
  c1.^2.*c3.*s3.^2+(-0.307200000000000000E5).*c1.^3.*c3.*s3.^2+ ...
  0.102400000000000000E5.*c1.^4.*c3.*s3.^2+(-0.292466962962962963E5) ...
  .*c1.^2.*c3.^2.*s3.^2+(-0.682666666666666667E4).*c1.^3.*c3.^2.* ...
  s3.^2+0.113777777777777778E4.*c1.^4.*c3.^2.*s3.^2+( ...
  -0.455111111111111111E4).*c1.^2.*c3.^3.*s3.^2+0.E-37.*c1.*s1.* ...
  s3.^2+0.E-37.*c1.*c3.*s1.*s3.^2+0.E-38.*c1.*c3.^2.*s1.*s3.^2+( ...
  -0.105130666666666667E6).*s1.^2.*s3.^2+0.460800000000000000E5.* ...
  c1.^2.*s1.^2.*s3.^2+(-0.525653333333333333E5).*c3.*s1.^2.*s3.^2+( ...
  -0.307200000000000000E5).*c1.*c3.*s1.^2.*s3.^2+ ...
  0.204800000000000000E5.*c1.^2.*c3.*s1.^2.*s3.^2+( ...
  -0.116811851851851852E5).*c3.^2.*s1.^2.*s3.^2+( ...
  -0.682666666666666667E4).*c1.*c3.^2.*s1.^2.*s3.^2+ ...
  0.227555555555555556E4.*c1.^2.*c3.^2.*s1.^2.*s3.^2+ ...
  0.230400000000000000E5.*s1.^4.*s3.^2+0.102400000000000000E5.*c3.* ...
  s1.^4.*s3.^2+0.113777777777777778E4.*c3.^2.*s1.^4.*s3.^2).^(-1),( ...
  0.427650666666666667E5.*c1.*s3+(-0.576000000000000000E4).*c1.^3.* ...
  s3+0.316225333333333333E5.*c1.*c3.*s3+0.768000000000000000E4.* ...
  c1.^2.*c3.*s3+(-0.256000000000000000E4).*c1.^3.*c3.*s3+ ...
  0.731167407407407407E4.*c1.*c3.^2.*s3+0.170666666666666667E4.* ...
  c1.^2.*c3.^2.*s3+(-0.284444444444444444E3).*c1.^3.*c3.^2.*s3+ ...
  0.113777777777777778E4.*c1.*c3.^3.*s3+(-0.394240000000000000E5).* ...
  s1.*s3+0.864000000000000000E4.*c1.^2.*s1.*s3+( ...
  -0.197120000000000000E5).*c3.*s1.*s3+(-0.576000000000000000E4).* ...
  c1.*c3.*s1.*s3+0.384000000000000000E4.*c1.^2.*c3.*s1.*s3+( ...
  -0.438044444444444444E4).*c3.^2.*s1.*s3+(-0.128000000000000000E4) ...
  .*c1.*c3.^2.*s1.*s3+0.426666666666666667E3.*c1.^2.*c3.^2.*s1.*s3+( ...
  -0.576000000000000000E4).*c1.*s1.^2.*s3+0.384000000000000000E4.* ...
  c3.*s1.^2.*s3+(-0.256000000000000000E4).*c1.*c3.*s1.^2.*s3+ ...
  0.853333333333333333E3.*c3.^2.*s1.^2.*s3+(-0.284444444444444444E3) ...
  .*c1.*c3.^2.*s1.^2.*s3+0.864000000000000000E4.*s1.^3.*s3+ ...
  0.384000000000000000E4.*c3.*s1.^3.*s3+0.426666666666666667E3.* ...
  c3.^2.*s1.^3.*s3).*(0.175621873777777778E7+0.E-37.*c1+( ...
  -0.236544000000000000E6).*c1.^2+0.129863203555555556E7.*c3+ ...
  0.315392000000000000E6.*c1.*c3+(-0.105130666666666667E6).*c1.^2.* ...
  c3+(-0.358315944691358025E6).*c3.^2+0.700871111111111111E5.*c1.* ...
  c3.^2+0.770228148148148148E5.*c1.^2.*c3.^2+( ...
  -0.440262272592592593E6).*c3.^3+(-0.118272000000000000E6).*c1.* ...
  c3.^3+0.394240000000000000E5.*c1.^2.*c3.^3+( ...
  -0.112599780740740741E6).*c3.^4+(-0.262826666666666667E5).*c1.* ...
  c3.^4+0.438044444444444444E4.*c1.^2.*c3.^4+( ...
  -0.175217777777777778E5).*c3.^5+0.E-39.*c1.*c3.^5+0.E-39.*c3.^6+ ...
  0.E-36.*s1+0.E-37.*c1.*s1+0.E-37.*c3.*s1+0.E-37.*c1.*c3.*s1+ ...
  0.E-37.*c3.^2.*s1+0.E-37.*c1.*c3.^2.*s1+0.E-37.*c3.^3.*s1+0.E-38.* ...
  c1.*c3.^3.*s1+0.E-38.*c3.^4.*s1+0.E-39.*c1.*c3.^4.*s1+0.E-39.* ...
  c3.^5.*s1+(-0.384885600000000000E6).*s1.^2+( ...
  -0.263220266666666667E6).*c3.*s1.^2+0.843654037037037037E5.* ...
  c3.^2.*s1.^2+0.941564888888888889E5.*c3.^3.*s1.^2+ ...
  0.224875111111111111E5.*c3.^4.*s1.^2+0.170666666666666667E4.* ...
  c3.^5.*s1.^2+(-0.171060266666666667E6).*c1.^2.*s3.^2+ ...
  0.230400000000000000E5.*c1.^4.*s3.^2+(-0.126490133333333333E6).* ...
  c1.^2.*c3.*s3.^2+(-0.307200000000000000E5).*c1.^3.*c3.*s3.^2+ ...
  0.102400000000000000E5.*c1.^4.*c3.*s3.^2+(-0.292466962962962963E5) ...
  .*c1.^2.*c3.^2.*s3.^2+(-0.682666666666666667E4).*c1.^3.*c3.^2.* ...
  s3.^2+0.113777777777777778E4.*c1.^4.*c3.^2.*s3.^2+( ...
  -0.455111111111111111E4).*c1.^2.*c3.^3.*s3.^2+0.E-37.*c1.*s1.* ...
  s3.^2+0.E-37.*c1.*c3.*s1.*s3.^2+0.E-38.*c1.*c3.^2.*s1.*s3.^2+( ...
  -0.105130666666666667E6).*s1.^2.*s3.^2+0.460800000000000000E5.* ...
  c1.^2.*s1.^2.*s3.^2+(-0.525653333333333333E5).*c3.*s1.^2.*s3.^2+( ...
  -0.307200000000000000E5).*c1.*c3.*s1.^2.*s3.^2+ ...
  0.204800000000000000E5.*c1.^2.*c3.*s1.^2.*s3.^2+( ...
  -0.116811851851851852E5).*c3.^2.*s1.^2.*s3.^2+( ...
  -0.682666666666666667E4).*c1.*c3.^2.*s1.^2.*s3.^2+ ...
  0.227555555555555556E4.*c1.^2.*c3.^2.*s1.^2.*s3.^2+ ...
  0.230400000000000000E5.*s1.^4.*s3.^2+0.102400000000000000E5.*c3.* ...
  s1.^4.*s3.^2+0.113777777777777778E4.*c3.^2.*s1.^4.*s3.^2).^(-1);(( ...
  -0.262826666666666667E5)+(-0.197120000000000000E5).*c1+( ...
  -0.438044444444444444E4).*c1.*c3+0.693570370370370370E4.*c3.^2+ ...
  0.739200000000000000E4.*c1.*c3.^2+0.164266666666666667E4.*c1.* ...
  c3.^3+0.109511111111111111E4.*c3.^4+0.213825333333333333E5.*s1+ ...
  0.384000000000000000E4.*c1.*s1+0.731167407407407407E4.*c3.*s1+ ...
  0.170666666666666667E4.*c1.*c3.*s1+(-0.744956111111111111E4).* ...
  c3.^2.*s1+(-0.125037037037037037E4).*c1.*c3.^2.*s1+( ...
  -0.274187777777777778E4).*c3.^3.*s1+(-0.640000000000000000E3).* ...
  c1.*c3.^3.*s1+(-0.213333333333333333E3).*c3.^4.*s1+( ...
  -0.711111111111111111E2).*c1.*c3.^4.*s1+0.576000000000000000E4.* ...
  s1.^2+0.256000000000000000E4.*c3.*s1.^2+(-0.187555555555555556E4) ...
  .*c3.^2.*s1.^2+(-0.960000000000000000E3).*c3.^3.*s1.^2+( ...
  -0.106666666666666667E3).*c3.^4.*s1.^2+0.256000000000000000E4.* ...
  c1.^2.*s3.^2+0.192000000000000000E4.*c1.^3.*s3.^2+ ...
  0.426666666666666667E3.*c1.^3.*c3.*s3.^2+0.284444444444444444E3.* ...
  c1.^2.*c3.^2.*s3.^2+(-0.170666666666666667E4).*c1.*s1.*s3.^2+( ...
  -0.128000000000000000E4).*c1.^2.*s1.*s3.^2+( ...
  -0.284444444444444444E3).*c1.^2.*c3.*s1.*s3.^2+( ...
  -0.189629629629629630E3).*c1.*c3.^2.*s1.*s3.^2+ ...
  0.192000000000000000E4.*c1.*s1.^2.*s3.^2+0.426666666666666667E3.* ...
  c1.*c3.*s1.^2.*s3.^2+(-0.128000000000000000E4).*s1.^3.*s3.^2+( ...
  -0.284444444444444444E3).*c3.*s1.^3.*s3.^2).*( ...
  0.175621873777777778E7+0.E-37.*c1+(-0.236544000000000000E6).* ...
  c1.^2+0.129863203555555556E7.*c3+0.315392000000000000E6.*c1.*c3+( ...
  -0.105130666666666667E6).*c1.^2.*c3+(-0.358315944691358025E6).* ...
  c3.^2+0.700871111111111111E5.*c1.*c3.^2+0.770228148148148148E5.* ...
  c1.^2.*c3.^2+(-0.440262272592592593E6).*c3.^3+( ...
  -0.118272000000000000E6).*c1.*c3.^3+0.394240000000000000E5.* ...
  c1.^2.*c3.^3+(-0.112599780740740741E6).*c3.^4+( ...
  -0.262826666666666667E5).*c1.*c3.^4+0.438044444444444444E4.* ...
  c1.^2.*c3.^4+(-0.175217777777777778E5).*c3.^5+0.E-39.*c1.*c3.^5+ ...
  0.E-39.*c3.^6+0.E-36.*s1+0.E-37.*c1.*s1+0.E-37.*c3.*s1+0.E-37.* ...
  c1.*c3.*s1+0.E-37.*c3.^2.*s1+0.E-37.*c1.*c3.^2.*s1+0.E-37.*c3.^3.* ...
  s1+0.E-38.*c1.*c3.^3.*s1+0.E-38.*c3.^4.*s1+0.E-39.*c1.*c3.^4.*s1+ ...
  0.E-39.*c3.^5.*s1+(-0.384885600000000000E6).*s1.^2+( ...
  -0.263220266666666667E6).*c3.*s1.^2+0.843654037037037037E5.* ...
  c3.^2.*s1.^2+0.941564888888888889E5.*c3.^3.*s1.^2+ ...
  0.224875111111111111E5.*c3.^4.*s1.^2+0.170666666666666667E4.* ...
  c3.^5.*s1.^2+(-0.171060266666666667E6).*c1.^2.*s3.^2+ ...
  0.230400000000000000E5.*c1.^4.*s3.^2+(-0.126490133333333333E6).* ...
  c1.^2.*c3.*s3.^2+(-0.307200000000000000E5).*c1.^3.*c3.*s3.^2+ ...
  0.102400000000000000E5.*c1.^4.*c3.*s3.^2+(-0.292466962962962963E5) ...
  .*c1.^2.*c3.^2.*s3.^2+(-0.682666666666666667E4).*c1.^3.*c3.^2.* ...
  s3.^2+0.113777777777777778E4.*c1.^4.*c3.^2.*s3.^2+( ...
  -0.455111111111111111E4).*c1.^2.*c3.^3.*s3.^2+0.E-37.*c1.*s1.* ...
  s3.^2+0.E-37.*c1.*c3.*s1.*s3.^2+0.E-38.*c1.*c3.^2.*s1.*s3.^2+( ...
  -0.105130666666666667E6).*s1.^2.*s3.^2+0.460800000000000000E5.* ...
  c1.^2.*s1.^2.*s3.^2+(-0.525653333333333333E5).*c3.*s1.^2.*s3.^2+( ...
  -0.307200000000000000E5).*c1.*c3.*s1.^2.*s3.^2+ ...
  0.204800000000000000E5.*c1.^2.*c3.*s1.^2.*s3.^2+( ...
  -0.116811851851851852E5).*c3.^2.*s1.^2.*s3.^2+( ...
  -0.682666666666666667E4).*c1.*c3.^2.*s1.^2.*s3.^2+ ...
  0.227555555555555556E4.*c1.^2.*c3.^2.*s1.^2.*s3.^2+ ...
  0.230400000000000000E5.*s1.^4.*s3.^2+0.102400000000000000E5.*c3.* ...
  s1.^4.*s3.^2+0.113777777777777778E4.*c3.^2.*s1.^4.*s3.^2).^(-1),( ...
  0.262826666666666667E5+0.197120000000000000E5.*c1+ ...
  0.438044444444444444E4.*c1.*c3+(-0.693570370370370370E4).*c3.^2+( ...
  -0.739200000000000000E4).*c1.*c3.^2+(-0.164266666666666667E4).* ...
  c1.*c3.^3+(-0.109511111111111111E4).*c3.^4+ ...
  0.213825333333333333E5.*s1+0.384000000000000000E4.*c1.*s1+ ...
  0.731167407407407407E4.*c3.*s1+0.170666666666666667E4.*c1.*c3.*s1+ ...
  (-0.744956111111111111E4).*c3.^2.*s1+(-0.125037037037037037E4).* ...
  c1.*c3.^2.*s1+(-0.274187777777777778E4).*c3.^3.*s1+( ...
  -0.640000000000000000E3).*c1.*c3.^3.*s1+(-0.213333333333333333E3) ...
  .*c3.^4.*s1+(-0.711111111111111111E2).*c1.*c3.^4.*s1+( ...
  -0.576000000000000000E4).*s1.^2+(-0.256000000000000000E4).*c3.* ...
  s1.^2+0.187555555555555556E4.*c3.^2.*s1.^2+ ...
  0.960000000000000000E3.*c3.^3.*s1.^2+0.106666666666666667E3.* ...
  c3.^4.*s1.^2+(-0.256000000000000000E4).*c1.^2.*s3.^2+( ...
  -0.192000000000000000E4).*c1.^3.*s3.^2+(-0.426666666666666667E3).* ...
  c1.^3.*c3.*s3.^2+(-0.284444444444444444E3).*c1.^2.*c3.^2.*s3.^2+( ...
  -0.170666666666666667E4).*c1.*s1.*s3.^2+(-0.128000000000000000E4) ...
  .*c1.^2.*s1.*s3.^2+(-0.284444444444444444E3).*c1.^2.*c3.*s1.* ...
  s3.^2+(-0.189629629629629630E3).*c1.*c3.^2.*s1.*s3.^2+( ...
  -0.192000000000000000E4).*c1.*s1.^2.*s3.^2+( ...
  -0.426666666666666667E3).*c1.*c3.*s1.^2.*s3.^2+( ...
  -0.128000000000000000E4).*s1.^3.*s3.^2+(-0.284444444444444444E3).* ...
  c3.*s1.^3.*s3.^2).*(0.175621873777777778E7+0.E-37.*c1+( ...
  -0.236544000000000000E6).*c1.^2+0.129863203555555556E7.*c3+ ...
  0.315392000000000000E6.*c1.*c3+(-0.105130666666666667E6).*c1.^2.* ...
  c3+(-0.358315944691358025E6).*c3.^2+0.700871111111111111E5.*c1.* ...
  c3.^2+0.770228148148148148E5.*c1.^2.*c3.^2+( ...
  -0.440262272592592593E6).*c3.^3+(-0.118272000000000000E6).*c1.* ...
  c3.^3+0.394240000000000000E5.*c1.^2.*c3.^3+( ...
  -0.112599780740740741E6).*c3.^4+(-0.262826666666666667E5).*c1.* ...
  c3.^4+0.438044444444444444E4.*c1.^2.*c3.^4+( ...
  -0.175217777777777778E5).*c3.^5+0.E-39.*c1.*c3.^5+0.E-39.*c3.^6+ ...
  0.E-36.*s1+0.E-37.*c1.*s1+0.E-37.*c3.*s1+0.E-37.*c1.*c3.*s1+ ...
  0.E-37.*c3.^2.*s1+0.E-37.*c1.*c3.^2.*s1+0.E-37.*c3.^3.*s1+0.E-38.* ...
  c1.*c3.^3.*s1+0.E-38.*c3.^4.*s1+0.E-39.*c1.*c3.^4.*s1+0.E-39.* ...
  c3.^5.*s1+(-0.384885600000000000E6).*s1.^2+( ...
  -0.263220266666666667E6).*c3.*s1.^2+0.843654037037037037E5.* ...
  c3.^2.*s1.^2+0.941564888888888889E5.*c3.^3.*s1.^2+ ...
  0.224875111111111111E5.*c3.^4.*s1.^2+0.170666666666666667E4.* ...
  c3.^5.*s1.^2+(-0.171060266666666667E6).*c1.^2.*s3.^2+ ...
  0.230400000000000000E5.*c1.^4.*s3.^2+(-0.126490133333333333E6).* ...
  c1.^2.*c3.*s3.^2+(-0.307200000000000000E5).*c1.^3.*c3.*s3.^2+ ...
  0.102400000000000000E5.*c1.^4.*c3.*s3.^2+(-0.292466962962962963E5) ...
  .*c1.^2.*c3.^2.*s3.^2+(-0.682666666666666667E4).*c1.^3.*c3.^2.* ...
  s3.^2+0.113777777777777778E4.*c1.^4.*c3.^2.*s3.^2+( ...
  -0.455111111111111111E4).*c1.^2.*c3.^3.*s3.^2+0.E-37.*c1.*s1.* ...
  s3.^2+0.E-37.*c1.*c3.*s1.*s3.^2+0.E-38.*c1.*c3.^2.*s1.*s3.^2+( ...
  -0.105130666666666667E6).*s1.^2.*s3.^2+0.460800000000000000E5.* ...
  c1.^2.*s1.^2.*s3.^2+(-0.525653333333333333E5).*c3.*s1.^2.*s3.^2+( ...
  -0.307200000000000000E5).*c1.*c3.*s1.^2.*s3.^2+ ...
  0.204800000000000000E5.*c1.^2.*c3.*s1.^2.*s3.^2+( ...
  -0.116811851851851852E5).*c3.^2.*s1.^2.*s3.^2+( ...
  -0.682666666666666667E4).*c1.*c3.^2.*s1.^2.*s3.^2+ ...
  0.227555555555555556E4.*c1.^2.*c3.^2.*s1.^2.*s3.^2+ ...
  0.230400000000000000E5.*s1.^4.*s3.^2+0.102400000000000000E5.*c3.* ...
  s1.^4.*s3.^2+0.113777777777777778E4.*c3.^2.*s1.^4.*s3.^2).^(-1),( ...
  0.906975585185185185E6+0.262826666666666667E6.*c1+ ...
  0.876088888888888889E5.*c3+0.584059259259259259E5.*c1.*c3+( ...
  -0.320647202469135802E6).*c3.^2+(-0.985600000000000000E5).*c1.* ...
  c3.^2+(-0.328533333333333333E5).*c3.^3+(-0.219022222222222222E5).* ...
  c1.*c3.^3+(-0.730074074074074074E4).*c3.^4+0.E-37.*s1+0.E-38.*c3.* ...
  s1+0.E-38.*c3.^2.*s1+0.E-38.*c3.^3.*s1+(-0.384000000000000000E5).* ...
  s1.^2+(-0.170666666666666667E5).*c3.*s1.^2+ ...
  0.125037037037037037E5.*c3.^2.*s1.^2+0.640000000000000000E4.* ...
  c3.^3.*s1.^2+0.711111111111111111E3.*c3.^4.*s1.^2+( ...
  -0.883417777777777778E5).*c1.^2.*s3.^2+(-0.256000000000000000E5).* ...
  c1.^3.*s3.^2+(-0.853333333333333333E4).*c1.^2.*c3.*s3.^2+( ...
  -0.568888888888888889E4).*c1.^3.*c3.*s3.^2+( ...
  -0.189629629629629630E4).*c1.^2.*c3.^2.*s3.^2+0.E-38.*c1.*s1.* ...
  s3.^2+(-0.438044444444444444E5).*s1.^2.*s3.^2+( ...
  -0.256000000000000000E5).*c1.*s1.^2.*s3.^2+( ...
  -0.568888888888888889E4).*c1.*c3.*s1.^2.*s3.^2).*( ...
  0.175621873777777778E7+0.E-37.*c1+(-0.236544000000000000E6).* ...
  c1.^2+0.129863203555555556E7.*c3+0.315392000000000000E6.*c1.*c3+( ...
  -0.105130666666666667E6).*c1.^2.*c3+(-0.358315944691358025E6).* ...
  c3.^2+0.700871111111111111E5.*c1.*c3.^2+0.770228148148148148E5.* ...
  c1.^2.*c3.^2+(-0.440262272592592593E6).*c3.^3+( ...
  -0.118272000000000000E6).*c1.*c3.^3+0.394240000000000000E5.* ...
  c1.^2.*c3.^3+(-0.112599780740740741E6).*c3.^4+( ...
  -0.262826666666666667E5).*c1.*c3.^4+0.438044444444444444E4.* ...
  c1.^2.*c3.^4+(-0.175217777777777778E5).*c3.^5+0.E-39.*c1.*c3.^5+ ...
  0.E-39.*c3.^6+0.E-36.*s1+0.E-37.*c1.*s1+0.E-37.*c3.*s1+0.E-37.* ...
  c1.*c3.*s1+0.E-37.*c3.^2.*s1+0.E-37.*c1.*c3.^2.*s1+0.E-37.*c3.^3.* ...
  s1+0.E-38.*c1.*c3.^3.*s1+0.E-38.*c3.^4.*s1+0.E-39.*c1.*c3.^4.*s1+ ...
  0.E-39.*c3.^5.*s1+(-0.384885600000000000E6).*s1.^2+( ...
  -0.263220266666666667E6).*c3.*s1.^2+0.843654037037037037E5.* ...
  c3.^2.*s1.^2+0.941564888888888889E5.*c3.^3.*s1.^2+ ...
  0.224875111111111111E5.*c3.^4.*s1.^2+0.170666666666666667E4.* ...
  c3.^5.*s1.^2+(-0.171060266666666667E6).*c1.^2.*s3.^2+ ...
  0.230400000000000000E5.*c1.^4.*s3.^2+(-0.126490133333333333E6).* ...
  c1.^2.*c3.*s3.^2+(-0.307200000000000000E5).*c1.^3.*c3.*s3.^2+ ...
  0.102400000000000000E5.*c1.^4.*c3.*s3.^2+(-0.292466962962962963E5) ...
  .*c1.^2.*c3.^2.*s3.^2+(-0.682666666666666667E4).*c1.^3.*c3.^2.* ...
  s3.^2+0.113777777777777778E4.*c1.^4.*c3.^2.*s3.^2+( ...
  -0.455111111111111111E4).*c1.^2.*c3.^3.*s3.^2+0.E-37.*c1.*s1.* ...
  s3.^2+0.E-37.*c1.*c3.*s1.*s3.^2+0.E-38.*c1.*c3.^2.*s1.*s3.^2+( ...
  -0.105130666666666667E6).*s1.^2.*s3.^2+0.460800000000000000E5.* ...
  c1.^2.*s1.^2.*s3.^2+(-0.525653333333333333E5).*c3.*s1.^2.*s3.^2+( ...
  -0.307200000000000000E5).*c1.*c3.*s1.^2.*s3.^2+ ...
  0.204800000000000000E5.*c1.^2.*c3.*s1.^2.*s3.^2+( ...
  -0.116811851851851852E5).*c3.^2.*s1.^2.*s3.^2+( ...
  -0.682666666666666667E4).*c1.*c3.^2.*s1.^2.*s3.^2+ ...
  0.227555555555555556E4.*c1.^2.*c3.^2.*s1.^2.*s3.^2+ ...
  0.230400000000000000E5.*s1.^4.*s3.^2+0.102400000000000000E5.*c3.* ...
  s1.^4.*s3.^2+0.113777777777777778E4.*c3.^2.*s1.^4.*s3.^2).^(-1),( ...
  0.E-38.*c1.*c3.*s3+0.E-38.*c1.^2.*c3.*s3+0.E-39.*c1.^2.*c3.^2.*s3+ ...
  0.E-39.*c1.*c3.^3.*s3+0.131413333333333333E5.*c3.*s1.*s3+( ...
  -0.618090000000000000E4).*c1.*c3.*s1.*s3+(-0.288000000000000000E4) ...
  .*c1.^2.*c3.*s1.*s3+(-0.329353333333333333E4).*c1.*c3.^2.*s1.*s3+( ...
  -0.128000000000000000E4).*c1.^2.*c3.^2.*s1.*s3+ ...
  0.146014814814814815E4.*c3.^3.*s1.*s3+(-0.426666666666666667E3).* ...
  c1.*c3.^3.*s1.*s3+(-0.142222222222222222E3).*c1.^2.*c3.^3.*s1.*s3+ ...
  0.E-38.*c3.*s1.^2.*s3+0.E-39.*c3.^2.*s1.^2.*s3+( ...
  -0.288000000000000000E4).*c3.*s1.^3.*s3+(-0.128000000000000000E4) ...
  .*c3.^2.*s1.^3.*s3+(-0.142222222222222222E3).*c3.^3.*s1.^3.*s3).*( ...
  0.175621873777777778E7+0.E-37.*c1+(-0.236544000000000000E6).* ...
  c1.^2+0.129863203555555556E7.*c3+0.315392000000000000E6.*c1.*c3+( ...
  -0.105130666666666667E6).*c1.^2.*c3+(-0.358315944691358025E6).* ...
  c3.^2+0.700871111111111111E5.*c1.*c3.^2+0.770228148148148148E5.* ...
  c1.^2.*c3.^2+(-0.440262272592592593E6).*c3.^3+( ...
  -0.118272000000000000E6).*c1.*c3.^3+0.394240000000000000E5.* ...
  c1.^2.*c3.^3+(-0.112599780740740741E6).*c3.^4+( ...
  -0.262826666666666667E5).*c1.*c3.^4+0.438044444444444444E4.* ...
  c1.^2.*c3.^4+(-0.175217777777777778E5).*c3.^5+0.E-39.*c1.*c3.^5+ ...
  0.E-39.*c3.^6+0.E-36.*s1+0.E-37.*c1.*s1+0.E-37.*c3.*s1+0.E-37.* ...
  c1.*c3.*s1+0.E-37.*c3.^2.*s1+0.E-37.*c1.*c3.^2.*s1+0.E-37.*c3.^3.* ...
  s1+0.E-38.*c1.*c3.^3.*s1+0.E-38.*c3.^4.*s1+0.E-39.*c1.*c3.^4.*s1+ ...
  0.E-39.*c3.^5.*s1+(-0.384885600000000000E6).*s1.^2+( ...
  -0.263220266666666667E6).*c3.*s1.^2+0.843654037037037037E5.* ...
  c3.^2.*s1.^2+0.941564888888888889E5.*c3.^3.*s1.^2+ ...
  0.224875111111111111E5.*c3.^4.*s1.^2+0.170666666666666667E4.* ...
  c3.^5.*s1.^2+(-0.171060266666666667E6).*c1.^2.*s3.^2+ ...
  0.230400000000000000E5.*c1.^4.*s3.^2+(-0.126490133333333333E6).* ...
  c1.^2.*c3.*s3.^2+(-0.307200000000000000E5).*c1.^3.*c3.*s3.^2+ ...
  0.102400000000000000E5.*c1.^4.*c3.*s3.^2+(-0.292466962962962963E5) ...
  .*c1.^2.*c3.^2.*s3.^2+(-0.682666666666666667E4).*c1.^3.*c3.^2.* ...
  s3.^2+0.113777777777777778E4.*c1.^4.*c3.^2.*s3.^2+( ...
  -0.455111111111111111E4).*c1.^2.*c3.^3.*s3.^2+0.E-37.*c1.*s1.* ...
  s3.^2+0.E-37.*c1.*c3.*s1.*s3.^2+0.E-38.*c1.*c3.^2.*s1.*s3.^2+( ...
  -0.105130666666666667E6).*s1.^2.*s3.^2+0.460800000000000000E5.* ...
  c1.^2.*s1.^2.*s3.^2+(-0.525653333333333333E5).*c3.*s1.^2.*s3.^2+( ...
  -0.307200000000000000E5).*c1.*c3.*s1.^2.*s3.^2+ ...
  0.204800000000000000E5.*c1.^2.*c3.*s1.^2.*s3.^2+( ...
  -0.116811851851851852E5).*c3.^2.*s1.^2.*s3.^2+( ...
  -0.682666666666666667E4).*c1.*c3.^2.*s1.^2.*s3.^2+ ...
  0.227555555555555556E4.*c1.^2.*c3.^2.*s1.^2.*s3.^2+ ...
  0.230400000000000000E5.*s1.^4.*s3.^2+0.102400000000000000E5.*c3.* ...
  s1.^4.*s3.^2+0.113777777777777778E4.*c3.^2.*s1.^4.*s3.^2).^(-1),( ...
  0.E-37.*c1.*s3+0.E-37.*c1.^2.*s3+0.E-38.*c1.^2.*c3.*s3+0.E-38.* ...
  c1.*c3.^2.*s3+(-0.262826666666666667E6).*s1.*s3+ ...
  0.123618000000000000E6.*c1.*s1.*s3+0.576000000000000000E5.*c1.^2.* ...
  s1.*s3+0.658706666666666667E5.*c1.*c3.*s1.*s3+ ...
  0.256000000000000000E5.*c1.^2.*c3.*s1.*s3+( ...
  -0.292029629629629630E5).*c3.^2.*s1.*s3+0.853333333333333333E4.* ...
  c1.*c3.^2.*s1.*s3+0.284444444444444444E4.*c1.^2.*c3.^2.*s1.*s3+ ...
  0.E-37.*s1.^2.*s3+0.E-38.*c3.*s1.^2.*s3+0.576000000000000000E5.* ...
  s1.^3.*s3+0.256000000000000000E5.*c3.*s1.^3.*s3+ ...
  0.284444444444444444E4.*c3.^2.*s1.^3.*s3).*( ...
  0.175621873777777778E7+0.E-37.*c1+(-0.236544000000000000E6).* ...
  c1.^2+0.129863203555555556E7.*c3+0.315392000000000000E6.*c1.*c3+( ...
  -0.105130666666666667E6).*c1.^2.*c3+(-0.358315944691358025E6).* ...
  c3.^2+0.700871111111111111E5.*c1.*c3.^2+0.770228148148148148E5.* ...
  c1.^2.*c3.^2+(-0.440262272592592593E6).*c3.^3+( ...
  -0.118272000000000000E6).*c1.*c3.^3+0.394240000000000000E5.* ...
  c1.^2.*c3.^3+(-0.112599780740740741E6).*c3.^4+( ...
  -0.262826666666666667E5).*c1.*c3.^4+0.438044444444444444E4.* ...
  c1.^2.*c3.^4+(-0.175217777777777778E5).*c3.^5+0.E-39.*c1.*c3.^5+ ...
  0.E-39.*c3.^6+0.E-36.*s1+0.E-37.*c1.*s1+0.E-37.*c3.*s1+0.E-37.* ...
  c1.*c3.*s1+0.E-37.*c3.^2.*s1+0.E-37.*c1.*c3.^2.*s1+0.E-37.*c3.^3.* ...
  s1+0.E-38.*c1.*c3.^3.*s1+0.E-38.*c3.^4.*s1+0.E-39.*c1.*c3.^4.*s1+ ...
  0.E-39.*c3.^5.*s1+(-0.384885600000000000E6).*s1.^2+( ...
  -0.263220266666666667E6).*c3.*s1.^2+0.843654037037037037E5.* ...
  c3.^2.*s1.^2+0.941564888888888889E5.*c3.^3.*s1.^2+ ...
  0.224875111111111111E5.*c3.^4.*s1.^2+0.170666666666666667E4.* ...
  c3.^5.*s1.^2+(-0.171060266666666667E6).*c1.^2.*s3.^2+ ...
  0.230400000000000000E5.*c1.^4.*s3.^2+(-0.126490133333333333E6).* ...
  c1.^2.*c3.*s3.^2+(-0.307200000000000000E5).*c1.^3.*c3.*s3.^2+ ...
  0.102400000000000000E5.*c1.^4.*c3.*s3.^2+(-0.292466962962962963E5) ...
  .*c1.^2.*c3.^2.*s3.^2+(-0.682666666666666667E4).*c1.^3.*c3.^2.* ...
  s3.^2+0.113777777777777778E4.*c1.^4.*c3.^2.*s3.^2+( ...
  -0.455111111111111111E4).*c1.^2.*c3.^3.*s3.^2+0.E-37.*c1.*s1.* ...
  s3.^2+0.E-37.*c1.*c3.*s1.*s3.^2+0.E-38.*c1.*c3.^2.*s1.*s3.^2+( ...
  -0.105130666666666667E6).*s1.^2.*s3.^2+0.460800000000000000E5.* ...
  c1.^2.*s1.^2.*s3.^2+(-0.525653333333333333E5).*c3.*s1.^2.*s3.^2+( ...
  -0.307200000000000000E5).*c1.*c3.*s1.^2.*s3.^2+ ...
  0.204800000000000000E5.*c1.^2.*c3.*s1.^2.*s3.^2+( ...
  -0.116811851851851852E5).*c3.^2.*s1.^2.*s3.^2+( ...
  -0.682666666666666667E4).*c1.*c3.^2.*s1.^2.*s3.^2+ ...
  0.227555555555555556E4.*c1.^2.*c3.^2.*s1.^2.*s3.^2+ ...
  0.230400000000000000E5.*s1.^4.*s3.^2+0.102400000000000000E5.*c3.* ...
  s1.^4.*s3.^2+0.113777777777777778E4.*c3.^2.*s1.^4.*s3.^2).^(-1);(( ...
  -0.213825333333333333E4).*c1.*c3.*s3+0.288000000000000000E3.* ...
  c1.^3.*c3.*s3+(-0.158112666666666667E4).*c1.*c3.^2.*s3+( ...
  -0.384000000000000000E3).*c1.^2.*c3.^2.*s3+ ...
  0.128000000000000000E3.*c1.^3.*c3.^2.*s3+(-0.365583703703703704E3) ...
  .*c1.*c3.^3.*s3+(-0.853333333333333333E2).*c1.^2.*c3.^3.*s3+ ...
  0.142222222222222222E2.*c1.^3.*c3.^3.*s3+(-0.568888888888888889E2) ...
  .*c1.*c3.^4.*s3+(-0.197120000000000000E4).*c3.*s1.*s3+ ...
  0.432000000000000000E3.*c1.^2.*c3.*s1.*s3+( ...
  -0.985600000000000000E3).*c3.^2.*s1.*s3+(-0.288000000000000000E3) ...
  .*c1.*c3.^2.*s1.*s3+0.192000000000000000E3.*c1.^2.*c3.^2.*s1.*s3+( ...
  -0.219022222222222222E3).*c3.^3.*s1.*s3+(-0.640000000000000000E2) ...
  .*c1.*c3.^3.*s1.*s3+0.213333333333333333E2.*c1.^2.*c3.^3.*s1.*s3+ ...
  0.288000000000000000E3.*c1.*c3.*s1.^2.*s3+( ...
  -0.192000000000000000E3).*c3.^2.*s1.^2.*s3+ ...
  0.128000000000000000E3.*c1.*c3.^2.*s1.^2.*s3+( ...
  -0.426666666666666667E2).*c3.^3.*s1.^2.*s3+ ...
  0.142222222222222222E2.*c1.*c3.^3.*s1.^2.*s3+ ...
  0.432000000000000000E3.*c3.*s1.^3.*s3+0.192000000000000000E3.* ...
  c3.^2.*s1.^3.*s3+0.213333333333333333E2.*c3.^3.*s1.^3.*s3).*( ...
  0.175621873777777778E7+0.E-37.*c1+(-0.236544000000000000E6).* ...
  c1.^2+0.129863203555555556E7.*c3+0.315392000000000000E6.*c1.*c3+( ...
  -0.105130666666666667E6).*c1.^2.*c3+(-0.358315944691358025E6).* ...
  c3.^2+0.700871111111111111E5.*c1.*c3.^2+0.770228148148148148E5.* ...
  c1.^2.*c3.^2+(-0.440262272592592593E6).*c3.^3+( ...
  -0.118272000000000000E6).*c1.*c3.^3+0.394240000000000000E5.* ...
  c1.^2.*c3.^3+(-0.112599780740740741E6).*c3.^4+( ...
  -0.262826666666666667E5).*c1.*c3.^4+0.438044444444444444E4.* ...
  c1.^2.*c3.^4+(-0.175217777777777778E5).*c3.^5+0.E-39.*c1.*c3.^5+ ...
  0.E-39.*c3.^6+0.E-36.*s1+0.E-37.*c1.*s1+0.E-37.*c3.*s1+0.E-37.* ...
  c1.*c3.*s1+0.E-37.*c3.^2.*s1+0.E-37.*c1.*c3.^2.*s1+0.E-37.*c3.^3.* ...
  s1+0.E-38.*c1.*c3.^3.*s1+0.E-38.*c3.^4.*s1+0.E-39.*c1.*c3.^4.*s1+ ...
  0.E-39.*c3.^5.*s1+(-0.384885600000000000E6).*s1.^2+( ...
  -0.263220266666666667E6).*c3.*s1.^2+0.843654037037037037E5.* ...
  c3.^2.*s1.^2+0.941564888888888889E5.*c3.^3.*s1.^2+ ...
  0.224875111111111111E5.*c3.^4.*s1.^2+0.170666666666666667E4.* ...
  c3.^5.*s1.^2+(-0.171060266666666667E6).*c1.^2.*s3.^2+ ...
  0.230400000000000000E5.*c1.^4.*s3.^2+(-0.126490133333333333E6).* ...
  c1.^2.*c3.*s3.^2+(-0.307200000000000000E5).*c1.^3.*c3.*s3.^2+ ...
  0.102400000000000000E5.*c1.^4.*c3.*s3.^2+(-0.292466962962962963E5) ...
  .*c1.^2.*c3.^2.*s3.^2+(-0.682666666666666667E4).*c1.^3.*c3.^2.* ...
  s3.^2+0.113777777777777778E4.*c1.^4.*c3.^2.*s3.^2+( ...
  -0.455111111111111111E4).*c1.^2.*c3.^3.*s3.^2+0.E-37.*c1.*s1.* ...
  s3.^2+0.E-37.*c1.*c3.*s1.*s3.^2+0.E-38.*c1.*c3.^2.*s1.*s3.^2+( ...
  -0.105130666666666667E6).*s1.^2.*s3.^2+0.460800000000000000E5.* ...
  c1.^2.*s1.^2.*s3.^2+(-0.525653333333333333E5).*c3.*s1.^2.*s3.^2+( ...
  -0.307200000000000000E5).*c1.*c3.*s1.^2.*s3.^2+ ...
  0.204800000000000000E5.*c1.^2.*c3.*s1.^2.*s3.^2+( ...
  -0.116811851851851852E5).*c3.^2.*s1.^2.*s3.^2+( ...
  -0.682666666666666667E4).*c1.*c3.^2.*s1.^2.*s3.^2+ ...
  0.227555555555555556E4.*c1.^2.*c3.^2.*s1.^2.*s3.^2+ ...
  0.230400000000000000E5.*s1.^4.*s3.^2+0.102400000000000000E5.*c3.* ...
  s1.^4.*s3.^2+0.113777777777777778E4.*c3.^2.*s1.^4.*s3.^2).^(-1),(( ...
  -0.213825333333333333E4).*c1.*c3.*s3+0.288000000000000000E3.* ...
  c1.^3.*c3.*s3+(-0.158112666666666667E4).*c1.*c3.^2.*s3+( ...
  -0.384000000000000000E3).*c1.^2.*c3.^2.*s3+ ...
  0.128000000000000000E3.*c1.^3.*c3.^2.*s3+(-0.365583703703703704E3) ...
  .*c1.*c3.^3.*s3+(-0.853333333333333333E2).*c1.^2.*c3.^3.*s3+ ...
  0.142222222222222222E2.*c1.^3.*c3.^3.*s3+(-0.568888888888888889E2) ...
  .*c1.*c3.^4.*s3+0.197120000000000000E4.*c3.*s1.*s3+( ...
  -0.432000000000000000E3).*c1.^2.*c3.*s1.*s3+ ...
  0.985600000000000000E3.*c3.^2.*s1.*s3+0.288000000000000000E3.*c1.* ...
  c3.^2.*s1.*s3+(-0.192000000000000000E3).*c1.^2.*c3.^2.*s1.*s3+ ...
  0.219022222222222222E3.*c3.^3.*s1.*s3+0.640000000000000000E2.*c1.* ...
  c3.^3.*s1.*s3+(-0.213333333333333333E2).*c1.^2.*c3.^3.*s1.*s3+ ...
  0.288000000000000000E3.*c1.*c3.*s1.^2.*s3+( ...
  -0.192000000000000000E3).*c3.^2.*s1.^2.*s3+ ...
  0.128000000000000000E3.*c1.*c3.^2.*s1.^2.*s3+( ...
  -0.426666666666666667E2).*c3.^3.*s1.^2.*s3+ ...
  0.142222222222222222E2.*c1.*c3.^3.*s1.^2.*s3+( ...
  -0.432000000000000000E3).*c3.*s1.^3.*s3+(-0.192000000000000000E3) ...
  .*c3.^2.*s1.^3.*s3+(-0.213333333333333333E2).*c3.^3.*s1.^3.*s3).*( ...
  0.175621873777777778E7+0.E-37.*c1+(-0.236544000000000000E6).* ...
  c1.^2+0.129863203555555556E7.*c3+0.315392000000000000E6.*c1.*c3+( ...
  -0.105130666666666667E6).*c1.^2.*c3+(-0.358315944691358025E6).* ...
  c3.^2+0.700871111111111111E5.*c1.*c3.^2+0.770228148148148148E5.* ...
  c1.^2.*c3.^2+(-0.440262272592592593E6).*c3.^3+( ...
  -0.118272000000000000E6).*c1.*c3.^3+0.394240000000000000E5.* ...
  c1.^2.*c3.^3+(-0.112599780740740741E6).*c3.^4+( ...
  -0.262826666666666667E5).*c1.*c3.^4+0.438044444444444444E4.* ...
  c1.^2.*c3.^4+(-0.175217777777777778E5).*c3.^5+0.E-39.*c1.*c3.^5+ ...
  0.E-39.*c3.^6+0.E-36.*s1+0.E-37.*c1.*s1+0.E-37.*c3.*s1+0.E-37.* ...
  c1.*c3.*s1+0.E-37.*c3.^2.*s1+0.E-37.*c1.*c3.^2.*s1+0.E-37.*c3.^3.* ...
  s1+0.E-38.*c1.*c3.^3.*s1+0.E-38.*c3.^4.*s1+0.E-39.*c1.*c3.^4.*s1+ ...
  0.E-39.*c3.^5.*s1+(-0.384885600000000000E6).*s1.^2+( ...
  -0.263220266666666667E6).*c3.*s1.^2+0.843654037037037037E5.* ...
  c3.^2.*s1.^2+0.941564888888888889E5.*c3.^3.*s1.^2+ ...
  0.224875111111111111E5.*c3.^4.*s1.^2+0.170666666666666667E4.* ...
  c3.^5.*s1.^2+(-0.171060266666666667E6).*c1.^2.*s3.^2+ ...
  0.230400000000000000E5.*c1.^4.*s3.^2+(-0.126490133333333333E6).* ...
  c1.^2.*c3.*s3.^2+(-0.307200000000000000E5).*c1.^3.*c3.*s3.^2+ ...
  0.102400000000000000E5.*c1.^4.*c3.*s3.^2+(-0.292466962962962963E5) ...
  .*c1.^2.*c3.^2.*s3.^2+(-0.682666666666666667E4).*c1.^3.*c3.^2.* ...
  s3.^2+0.113777777777777778E4.*c1.^4.*c3.^2.*s3.^2+( ...
  -0.455111111111111111E4).*c1.^2.*c3.^3.*s3.^2+0.E-37.*c1.*s1.* ...
  s3.^2+0.E-37.*c1.*c3.*s1.*s3.^2+0.E-38.*c1.*c3.^2.*s1.*s3.^2+( ...
  -0.105130666666666667E6).*s1.^2.*s3.^2+0.460800000000000000E5.* ...
  c1.^2.*s1.^2.*s3.^2+(-0.525653333333333333E5).*c3.*s1.^2.*s3.^2+( ...
  -0.307200000000000000E5).*c1.*c3.*s1.^2.*s3.^2+ ...
  0.204800000000000000E5.*c1.^2.*c3.*s1.^2.*s3.^2+( ...
  -0.116811851851851852E5).*c3.^2.*s1.^2.*s3.^2+( ...
  -0.682666666666666667E4).*c1.*c3.^2.*s1.^2.*s3.^2+ ...
  0.227555555555555556E4.*c1.^2.*c3.^2.*s1.^2.*s3.^2+ ...
  0.230400000000000000E5.*s1.^4.*s3.^2+0.102400000000000000E5.*c3.* ...
  s1.^4.*s3.^2+0.113777777777777778E4.*c3.^2.*s1.^4.*s3.^2).^(-1),( ...
  0.E-38.*c1.*c3.*s3+0.E-38.*c1.^2.*c3.*s3+0.E-39.*c1.^2.*c3.^2.*s3+ ...
  0.E-39.*c1.*c3.^3.*s3+0.131413333333333333E5.*c3.*s1.*s3+( ...
  -0.618090000000000000E4).*c1.*c3.*s1.*s3+(-0.288000000000000000E4) ...
  .*c1.^2.*c3.*s1.*s3+(-0.329353333333333333E4).*c1.*c3.^2.*s1.*s3+( ...
  -0.128000000000000000E4).*c1.^2.*c3.^2.*s1.*s3+ ...
  0.146014814814814815E4.*c3.^3.*s1.*s3+(-0.426666666666666667E3).* ...
  c1.*c3.^3.*s1.*s3+(-0.142222222222222222E3).*c1.^2.*c3.^3.*s1.*s3+ ...
  0.E-38.*c3.*s1.^2.*s3+0.E-39.*c3.^2.*s1.^2.*s3+( ...
  -0.288000000000000000E4).*c3.*s1.^3.*s3+(-0.128000000000000000E4) ...
  .*c3.^2.*s1.^3.*s3+(-0.142222222222222222E3).*c3.^3.*s1.^3.*s3).*( ...
  0.175621873777777778E7+0.E-37.*c1+(-0.236544000000000000E6).* ...
  c1.^2+0.129863203555555556E7.*c3+0.315392000000000000E6.*c1.*c3+( ...
  -0.105130666666666667E6).*c1.^2.*c3+(-0.358315944691358025E6).* ...
  c3.^2+0.700871111111111111E5.*c1.*c3.^2+0.770228148148148148E5.* ...
  c1.^2.*c3.^2+(-0.440262272592592593E6).*c3.^3+( ...
  -0.118272000000000000E6).*c1.*c3.^3+0.394240000000000000E5.* ...
  c1.^2.*c3.^3+(-0.112599780740740741E6).*c3.^4+( ...
  -0.262826666666666667E5).*c1.*c3.^4+0.438044444444444444E4.* ...
  c1.^2.*c3.^4+(-0.175217777777777778E5).*c3.^5+0.E-39.*c1.*c3.^5+ ...
  0.E-39.*c3.^6+0.E-36.*s1+0.E-37.*c1.*s1+0.E-37.*c3.*s1+0.E-37.* ...
  c1.*c3.*s1+0.E-37.*c3.^2.*s1+0.E-37.*c1.*c3.^2.*s1+0.E-37.*c3.^3.* ...
  s1+0.E-38.*c1.*c3.^3.*s1+0.E-38.*c3.^4.*s1+0.E-39.*c1.*c3.^4.*s1+ ...
  0.E-39.*c3.^5.*s1+(-0.384885600000000000E6).*s1.^2+( ...
  -0.263220266666666667E6).*c3.*s1.^2+0.843654037037037037E5.* ...
  c3.^2.*s1.^2+0.941564888888888889E5.*c3.^3.*s1.^2+ ...
  0.224875111111111111E5.*c3.^4.*s1.^2+0.170666666666666667E4.* ...
  c3.^5.*s1.^2+(-0.171060266666666667E6).*c1.^2.*s3.^2+ ...
  0.230400000000000000E5.*c1.^4.*s3.^2+(-0.126490133333333333E6).* ...
  c1.^2.*c3.*s3.^2+(-0.307200000000000000E5).*c1.^3.*c3.*s3.^2+ ...
  0.102400000000000000E5.*c1.^4.*c3.*s3.^2+(-0.292466962962962963E5) ...
  .*c1.^2.*c3.^2.*s3.^2+(-0.682666666666666667E4).*c1.^3.*c3.^2.* ...
  s3.^2+0.113777777777777778E4.*c1.^4.*c3.^2.*s3.^2+( ...
  -0.455111111111111111E4).*c1.^2.*c3.^3.*s3.^2+0.E-37.*c1.*s1.* ...
  s3.^2+0.E-37.*c1.*c3.*s1.*s3.^2+0.E-38.*c1.*c3.^2.*s1.*s3.^2+( ...
  -0.105130666666666667E6).*s1.^2.*s3.^2+0.460800000000000000E5.* ...
  c1.^2.*s1.^2.*s3.^2+(-0.525653333333333333E5).*c3.*s1.^2.*s3.^2+( ...
  -0.307200000000000000E5).*c1.*c3.*s1.^2.*s3.^2+ ...
  0.204800000000000000E5.*c1.^2.*c3.*s1.^2.*s3.^2+( ...
  -0.116811851851851852E5).*c3.^2.*s1.^2.*s3.^2+( ...
  -0.682666666666666667E4).*c1.*c3.^2.*s1.^2.*s3.^2+ ...
  0.227555555555555556E4.*c1.^2.*c3.^2.*s1.^2.*s3.^2+ ...
  0.230400000000000000E5.*s1.^4.*s3.^2+0.102400000000000000E5.*c3.* ...
  s1.^4.*s3.^2+0.113777777777777778E4.*c3.^2.*s1.^4.*s3.^2).^(-1),( ...
  0.439054684444444444E5+0.E-38.*c1+(-0.591360000000000000E4).* ...
  c1.^2+0.324658008888888889E5.*c3+0.788480000000000000E4.*c1.*c3+( ...
  -0.262826666666666667E4).*c1.^2.*c3+0.750665204938271605E4.*c3.^2+ ...
  0.175217777777777778E4.*c1.*c3.^2+(-0.292029629629629630E3).* ...
  c1.^2.*c3.^2+0.116811851851851852E4.*c3.^3+0.E-40.*c1.*c3.^3+ ...
  0.E-40.*c3.^4+0.E-38.*s1+0.E-38.*c1.*s1+0.E-38.*c3.*s1+0.E-39.* ...
  c1.*c3.*s1+0.E-39.*c3.^2.*s1+0.E-40.*c1.*c3.^2.*s1+0.E-40.*c3.^3.* ...
  s1+(-0.962214000000000000E4).*s1.^2+(-0.658050666666666667E4).* ...
  c3.*s1.^2+(-0.149916740740740741E4).*c3.^2.*s1.^2+( ...
  -0.113777777777777778E3).*c3.^3.*s1.^2+(-0.427650666666666667E4).* ...
  c1.^2.*s3.^2+0.576000000000000000E3.*c1.^4.*s3.^2+( ...
  -0.316225333333333333E4).*c1.^2.*c3.*s3.^2+( ...
  -0.768000000000000000E3).*c1.^3.*c3.*s3.^2+ ...
  0.256000000000000000E3.*c1.^4.*c3.*s3.^2+(-0.731167407407407407E3) ...
  .*c1.^2.*c3.^2.*s3.^2+(-0.170666666666666667E3).*c1.^3.*c3.^2.* ...
  s3.^2+0.284444444444444444E2.*c1.^4.*c3.^2.*s3.^2+( ...
  -0.113777777777777778E3).*c1.^2.*c3.^3.*s3.^2+0.E-39.*c1.*s1.* ...
  s3.^2+0.E-39.*c1.*c3.*s1.*s3.^2+0.E-40.*c1.*c3.^2.*s1.*s3.^2+( ...
  -0.262826666666666667E4).*s1.^2.*s3.^2+0.115200000000000000E4.* ...
  c1.^2.*s1.^2.*s3.^2+(-0.131413333333333333E4).*c3.*s1.^2.*s3.^2+( ...
  -0.768000000000000000E3).*c1.*c3.*s1.^2.*s3.^2+ ...
  0.512000000000000000E3.*c1.^2.*c3.*s1.^2.*s3.^2+( ...
  -0.292029629629629630E3).*c3.^2.*s1.^2.*s3.^2+( ...
  -0.170666666666666667E3).*c1.*c3.^2.*s1.^2.*s3.^2+ ...
  0.568888888888888889E2.*c1.^2.*c3.^2.*s1.^2.*s3.^2+ ...
  0.576000000000000000E3.*s1.^4.*s3.^2+0.256000000000000000E3.*c3.* ...
  s1.^4.*s3.^2+0.284444444444444444E2.*c3.^2.*s1.^4.*s3.^2).*( ...
  0.175621873777777778E7+0.E-37.*c1+(-0.236544000000000000E6).* ...
  c1.^2+0.129863203555555556E7.*c3+0.315392000000000000E6.*c1.*c3+( ...
  -0.105130666666666667E6).*c1.^2.*c3+(-0.358315944691358025E6).* ...
  c3.^2+0.700871111111111111E5.*c1.*c3.^2+0.770228148148148148E5.* ...
  c1.^2.*c3.^2+(-0.440262272592592593E6).*c3.^3+( ...
  -0.118272000000000000E6).*c1.*c3.^3+0.394240000000000000E5.* ...
  c1.^2.*c3.^3+(-0.112599780740740741E6).*c3.^4+( ...
  -0.262826666666666667E5).*c1.*c3.^4+0.438044444444444444E4.* ...
  c1.^2.*c3.^4+(-0.175217777777777778E5).*c3.^5+0.E-39.*c1.*c3.^5+ ...
  0.E-39.*c3.^6+0.E-36.*s1+0.E-37.*c1.*s1+0.E-37.*c3.*s1+0.E-37.* ...
  c1.*c3.*s1+0.E-37.*c3.^2.*s1+0.E-37.*c1.*c3.^2.*s1+0.E-37.*c3.^3.* ...
  s1+0.E-38.*c1.*c3.^3.*s1+0.E-38.*c3.^4.*s1+0.E-39.*c1.*c3.^4.*s1+ ...
  0.E-39.*c3.^5.*s1+(-0.384885600000000000E6).*s1.^2+( ...
  -0.263220266666666667E6).*c3.*s1.^2+0.843654037037037037E5.* ...
  c3.^2.*s1.^2+0.941564888888888889E5.*c3.^3.*s1.^2+ ...
  0.224875111111111111E5.*c3.^4.*s1.^2+0.170666666666666667E4.* ...
  c3.^5.*s1.^2+(-0.171060266666666667E6).*c1.^2.*s3.^2+ ...
  0.230400000000000000E5.*c1.^4.*s3.^2+(-0.126490133333333333E6).* ...
  c1.^2.*c3.*s3.^2+(-0.307200000000000000E5).*c1.^3.*c3.*s3.^2+ ...
  0.102400000000000000E5.*c1.^4.*c3.*s3.^2+(-0.292466962962962963E5) ...
  .*c1.^2.*c3.^2.*s3.^2+(-0.682666666666666667E4).*c1.^3.*c3.^2.* ...
  s3.^2+0.113777777777777778E4.*c1.^4.*c3.^2.*s3.^2+( ...
  -0.455111111111111111E4).*c1.^2.*c3.^3.*s3.^2+0.E-37.*c1.*s1.* ...
  s3.^2+0.E-37.*c1.*c3.*s1.*s3.^2+0.E-38.*c1.*c3.^2.*s1.*s3.^2+( ...
  -0.105130666666666667E6).*s1.^2.*s3.^2+0.460800000000000000E5.* ...
  c1.^2.*s1.^2.*s3.^2+(-0.525653333333333333E5).*c3.*s1.^2.*s3.^2+( ...
  -0.307200000000000000E5).*c1.*c3.*s1.^2.*s3.^2+ ...
  0.204800000000000000E5.*c1.^2.*c3.*s1.^2.*s3.^2+( ...
  -0.116811851851851852E5).*c3.^2.*s1.^2.*s3.^2+( ...
  -0.682666666666666667E4).*c1.*c3.^2.*s1.^2.*s3.^2+ ...
  0.227555555555555556E4.*c1.^2.*c3.^2.*s1.^2.*s3.^2+ ...
  0.230400000000000000E5.*s1.^4.*s3.^2+0.102400000000000000E5.*c3.* ...
  s1.^4.*s3.^2+0.113777777777777778E4.*c3.^2.*s1.^4.*s3.^2).^(-1),(( ...
  -0.329291013333333333E6).*c3+0.E-37.*c1.*c3+ ...
  0.443520000000000000E5.*c1.^2.*c3+(-0.243493506666666667E6).* ...
  c3.^2+(-0.591360000000000000E5).*c1.*c3.^2+ ...
  0.197120000000000000E5.*c1.^2.*c3.^2+(-0.562998903703703704E5).* ...
  c3.^3+(-0.131413333333333333E5).*c1.*c3.^3+ ...
  0.219022222222222222E4.*c1.^2.*c3.^3+(-0.876088888888888889E4).* ...
  c3.^4+0.E-39.*c1.*c3.^4+0.E-39.*c3.^5+0.E-37.*c3.*s1+0.E-38.*c1.* ...
  c3.*s1+0.E-38.*c3.^2.*s1+0.E-38.*c1.*c3.^2.*s1+0.E-38.*c3.^3.*s1+ ...
  0.E-39.*c1.*c3.^3.*s1+0.E-39.*c3.^4.*s1+0.721660500000000000E5.* ...
  c3.*s1.^2+0.493538000000000000E5.*c3.^2.*s1.^2+ ...
  0.112437555555555556E5.*c3.^3.*s1.^2+0.853333333333333333E3.* ...
  c3.^4.*s1.^2).*(0.175621873777777778E7+0.E-37.*c1+( ...
  -0.236544000000000000E6).*c1.^2+0.129863203555555556E7.*c3+ ...
  0.315392000000000000E6.*c1.*c3+(-0.105130666666666667E6).*c1.^2.* ...
  c3+(-0.358315944691358025E6).*c3.^2+0.700871111111111111E5.*c1.* ...
  c3.^2+0.770228148148148148E5.*c1.^2.*c3.^2+( ...
  -0.440262272592592593E6).*c3.^3+(-0.118272000000000000E6).*c1.* ...
  c3.^3+0.394240000000000000E5.*c1.^2.*c3.^3+( ...
  -0.112599780740740741E6).*c3.^4+(-0.262826666666666667E5).*c1.* ...
  c3.^4+0.438044444444444444E4.*c1.^2.*c3.^4+( ...
  -0.175217777777777778E5).*c3.^5+0.E-39.*c1.*c3.^5+0.E-39.*c3.^6+ ...
  0.E-36.*s1+0.E-37.*c1.*s1+0.E-37.*c3.*s1+0.E-37.*c1.*c3.*s1+ ...
  0.E-37.*c3.^2.*s1+0.E-37.*c1.*c3.^2.*s1+0.E-37.*c3.^3.*s1+0.E-38.* ...
  c1.*c3.^3.*s1+0.E-38.*c3.^4.*s1+0.E-39.*c1.*c3.^4.*s1+0.E-39.* ...
  c3.^5.*s1+(-0.384885600000000000E6).*s1.^2+( ...
  -0.263220266666666667E6).*c3.*s1.^2+0.843654037037037037E5.* ...
  c3.^2.*s1.^2+0.941564888888888889E5.*c3.^3.*s1.^2+ ...
  0.224875111111111111E5.*c3.^4.*s1.^2+0.170666666666666667E4.* ...
  c3.^5.*s1.^2+(-0.171060266666666667E6).*c1.^2.*s3.^2+ ...
  0.230400000000000000E5.*c1.^4.*s3.^2+(-0.126490133333333333E6).* ...
  c1.^2.*c3.*s3.^2+(-0.307200000000000000E5).*c1.^3.*c3.*s3.^2+ ...
  0.102400000000000000E5.*c1.^4.*c3.*s3.^2+(-0.292466962962962963E5) ...
  .*c1.^2.*c3.^2.*s3.^2+(-0.682666666666666667E4).*c1.^3.*c3.^2.* ...
  s3.^2+0.113777777777777778E4.*c1.^4.*c3.^2.*s3.^2+( ...
  -0.455111111111111111E4).*c1.^2.*c3.^3.*s3.^2+0.E-37.*c1.*s1.* ...
  s3.^2+0.E-37.*c1.*c3.*s1.*s3.^2+0.E-38.*c1.*c3.^2.*s1.*s3.^2+( ...
  -0.105130666666666667E6).*s1.^2.*s3.^2+0.460800000000000000E5.* ...
  c1.^2.*s1.^2.*s3.^2+(-0.525653333333333333E5).*c3.*s1.^2.*s3.^2+( ...
  -0.307200000000000000E5).*c1.*c3.*s1.^2.*s3.^2+ ...
  0.204800000000000000E5.*c1.^2.*c3.*s1.^2.*s3.^2+( ...
  -0.116811851851851852E5).*c3.^2.*s1.^2.*s3.^2+( ...
  -0.682666666666666667E4).*c1.*c3.^2.*s1.^2.*s3.^2+ ...
  0.227555555555555556E4.*c1.^2.*c3.^2.*s1.^2.*s3.^2+ ...
  0.230400000000000000E5.*s1.^4.*s3.^2+0.102400000000000000E5.*c3.* ...
  s1.^4.*s3.^2+0.113777777777777778E4.*c3.^2.*s1.^4.*s3.^2).^(-1);( ...
  0.427650666666666667E5.*c1.*s3+(-0.576000000000000000E4).*c1.^3.* ...
  s3+0.316225333333333333E5.*c1.*c3.*s3+0.768000000000000000E4.* ...
  c1.^2.*c3.*s3+(-0.256000000000000000E4).*c1.^3.*c3.*s3+ ...
  0.731167407407407407E4.*c1.*c3.^2.*s3+0.170666666666666667E4.* ...
  c1.^2.*c3.^2.*s3+(-0.284444444444444444E3).*c1.^3.*c3.^2.*s3+ ...
  0.113777777777777778E4.*c1.*c3.^3.*s3+0.394240000000000000E5.*s1.* ...
  s3+(-0.864000000000000000E4).*c1.^2.*s1.*s3+ ...
  0.197120000000000000E5.*c3.*s1.*s3+0.576000000000000000E4.*c1.* ...
  c3.*s1.*s3+(-0.384000000000000000E4).*c1.^2.*c3.*s1.*s3+ ...
  0.438044444444444444E4.*c3.^2.*s1.*s3+0.128000000000000000E4.*c1.* ...
  c3.^2.*s1.*s3+(-0.426666666666666667E3).*c1.^2.*c3.^2.*s1.*s3+( ...
  -0.576000000000000000E4).*c1.*s1.^2.*s3+0.384000000000000000E4.* ...
  c3.*s1.^2.*s3+(-0.256000000000000000E4).*c1.*c3.*s1.^2.*s3+ ...
  0.853333333333333333E3.*c3.^2.*s1.^2.*s3+(-0.284444444444444444E3) ...
  .*c1.*c3.^2.*s1.^2.*s3+(-0.864000000000000000E4).*s1.^3.*s3+( ...
  -0.384000000000000000E4).*c3.*s1.^3.*s3+(-0.426666666666666667E3) ...
  .*c3.^2.*s1.^3.*s3).*(0.175621873777777778E7+0.E-37.*c1+( ...
  -0.236544000000000000E6).*c1.^2+0.129863203555555556E7.*c3+ ...
  0.315392000000000000E6.*c1.*c3+(-0.105130666666666667E6).*c1.^2.* ...
  c3+(-0.358315944691358025E6).*c3.^2+0.700871111111111111E5.*c1.* ...
  c3.^2+0.770228148148148148E5.*c1.^2.*c3.^2+( ...
  -0.440262272592592593E6).*c3.^3+(-0.118272000000000000E6).*c1.* ...
  c3.^3+0.394240000000000000E5.*c1.^2.*c3.^3+( ...
  -0.112599780740740741E6).*c3.^4+(-0.262826666666666667E5).*c1.* ...
  c3.^4+0.438044444444444444E4.*c1.^2.*c3.^4+( ...
  -0.175217777777777778E5).*c3.^5+0.E-39.*c1.*c3.^5+0.E-39.*c3.^6+ ...
  0.E-36.*s1+0.E-37.*c1.*s1+0.E-37.*c3.*s1+0.E-37.*c1.*c3.*s1+ ...
  0.E-37.*c3.^2.*s1+0.E-37.*c1.*c3.^2.*s1+0.E-37.*c3.^3.*s1+0.E-38.* ...
  c1.*c3.^3.*s1+0.E-38.*c3.^4.*s1+0.E-39.*c1.*c3.^4.*s1+0.E-39.* ...
  c3.^5.*s1+(-0.384885600000000000E6).*s1.^2+( ...
  -0.263220266666666667E6).*c3.*s1.^2+0.843654037037037037E5.* ...
  c3.^2.*s1.^2+0.941564888888888889E5.*c3.^3.*s1.^2+ ...
  0.224875111111111111E5.*c3.^4.*s1.^2+0.170666666666666667E4.* ...
  c3.^5.*s1.^2+(-0.171060266666666667E6).*c1.^2.*s3.^2+ ...
  0.230400000000000000E5.*c1.^4.*s3.^2+(-0.126490133333333333E6).* ...
  c1.^2.*c3.*s3.^2+(-0.307200000000000000E5).*c1.^3.*c3.*s3.^2+ ...
  0.102400000000000000E5.*c1.^4.*c3.*s3.^2+(-0.292466962962962963E5) ...
  .*c1.^2.*c3.^2.*s3.^2+(-0.682666666666666667E4).*c1.^3.*c3.^2.* ...
  s3.^2+0.113777777777777778E4.*c1.^4.*c3.^2.*s3.^2+( ...
  -0.455111111111111111E4).*c1.^2.*c3.^3.*s3.^2+0.E-37.*c1.*s1.* ...
  s3.^2+0.E-37.*c1.*c3.*s1.*s3.^2+0.E-38.*c1.*c3.^2.*s1.*s3.^2+( ...
  -0.105130666666666667E6).*s1.^2.*s3.^2+0.460800000000000000E5.* ...
  c1.^2.*s1.^2.*s3.^2+(-0.525653333333333333E5).*c3.*s1.^2.*s3.^2+( ...
  -0.307200000000000000E5).*c1.*c3.*s1.^2.*s3.^2+ ...
  0.204800000000000000E5.*c1.^2.*c3.*s1.^2.*s3.^2+( ...
  -0.116811851851851852E5).*c3.^2.*s1.^2.*s3.^2+( ...
  -0.682666666666666667E4).*c1.*c3.^2.*s1.^2.*s3.^2+ ...
  0.227555555555555556E4.*c1.^2.*c3.^2.*s1.^2.*s3.^2+ ...
  0.230400000000000000E5.*s1.^4.*s3.^2+0.102400000000000000E5.*c3.* ...
  s1.^4.*s3.^2+0.113777777777777778E4.*c3.^2.*s1.^4.*s3.^2).^(-1),( ...
  0.427650666666666667E5.*c1.*s3+(-0.576000000000000000E4).*c1.^3.* ...
  s3+0.316225333333333333E5.*c1.*c3.*s3+0.768000000000000000E4.* ...
  c1.^2.*c3.*s3+(-0.256000000000000000E4).*c1.^3.*c3.*s3+ ...
  0.731167407407407407E4.*c1.*c3.^2.*s3+0.170666666666666667E4.* ...
  c1.^2.*c3.^2.*s3+(-0.284444444444444444E3).*c1.^3.*c3.^2.*s3+ ...
  0.113777777777777778E4.*c1.*c3.^3.*s3+(-0.394240000000000000E5).* ...
  s1.*s3+0.864000000000000000E4.*c1.^2.*s1.*s3+( ...
  -0.197120000000000000E5).*c3.*s1.*s3+(-0.576000000000000000E4).* ...
  c1.*c3.*s1.*s3+0.384000000000000000E4.*c1.^2.*c3.*s1.*s3+( ...
  -0.438044444444444444E4).*c3.^2.*s1.*s3+(-0.128000000000000000E4) ...
  .*c1.*c3.^2.*s1.*s3+0.426666666666666667E3.*c1.^2.*c3.^2.*s1.*s3+( ...
  -0.576000000000000000E4).*c1.*s1.^2.*s3+0.384000000000000000E4.* ...
  c3.*s1.^2.*s3+(-0.256000000000000000E4).*c1.*c3.*s1.^2.*s3+ ...
  0.853333333333333333E3.*c3.^2.*s1.^2.*s3+(-0.284444444444444444E3) ...
  .*c1.*c3.^2.*s1.^2.*s3+0.864000000000000000E4.*s1.^3.*s3+ ...
  0.384000000000000000E4.*c3.*s1.^3.*s3+0.426666666666666667E3.* ...
  c3.^2.*s1.^3.*s3).*(0.175621873777777778E7+0.E-37.*c1+( ...
  -0.236544000000000000E6).*c1.^2+0.129863203555555556E7.*c3+ ...
  0.315392000000000000E6.*c1.*c3+(-0.105130666666666667E6).*c1.^2.* ...
  c3+(-0.358315944691358025E6).*c3.^2+0.700871111111111111E5.*c1.* ...
  c3.^2+0.770228148148148148E5.*c1.^2.*c3.^2+( ...
  -0.440262272592592593E6).*c3.^3+(-0.118272000000000000E6).*c1.* ...
  c3.^3+0.394240000000000000E5.*c1.^2.*c3.^3+( ...
  -0.112599780740740741E6).*c3.^4+(-0.262826666666666667E5).*c1.* ...
  c3.^4+0.438044444444444444E4.*c1.^2.*c3.^4+( ...
  -0.175217777777777778E5).*c3.^5+0.E-39.*c1.*c3.^5+0.E-39.*c3.^6+ ...
  0.E-36.*s1+0.E-37.*c1.*s1+0.E-37.*c3.*s1+0.E-37.*c1.*c3.*s1+ ...
  0.E-37.*c3.^2.*s1+0.E-37.*c1.*c3.^2.*s1+0.E-37.*c3.^3.*s1+0.E-38.* ...
  c1.*c3.^3.*s1+0.E-38.*c3.^4.*s1+0.E-39.*c1.*c3.^4.*s1+0.E-39.* ...
  c3.^5.*s1+(-0.384885600000000000E6).*s1.^2+( ...
  -0.263220266666666667E6).*c3.*s1.^2+0.843654037037037037E5.* ...
  c3.^2.*s1.^2+0.941564888888888889E5.*c3.^3.*s1.^2+ ...
  0.224875111111111111E5.*c3.^4.*s1.^2+0.170666666666666667E4.* ...
  c3.^5.*s1.^2+(-0.171060266666666667E6).*c1.^2.*s3.^2+ ...
  0.230400000000000000E5.*c1.^4.*s3.^2+(-0.126490133333333333E6).* ...
  c1.^2.*c3.*s3.^2+(-0.307200000000000000E5).*c1.^3.*c3.*s3.^2+ ...
  0.102400000000000000E5.*c1.^4.*c3.*s3.^2+(-0.292466962962962963E5) ...
  .*c1.^2.*c3.^2.*s3.^2+(-0.682666666666666667E4).*c1.^3.*c3.^2.* ...
  s3.^2+0.113777777777777778E4.*c1.^4.*c3.^2.*s3.^2+( ...
  -0.455111111111111111E4).*c1.^2.*c3.^3.*s3.^2+0.E-37.*c1.*s1.* ...
  s3.^2+0.E-37.*c1.*c3.*s1.*s3.^2+0.E-38.*c1.*c3.^2.*s1.*s3.^2+( ...
  -0.105130666666666667E6).*s1.^2.*s3.^2+0.460800000000000000E5.* ...
  c1.^2.*s1.^2.*s3.^2+(-0.525653333333333333E5).*c3.*s1.^2.*s3.^2+( ...
  -0.307200000000000000E5).*c1.*c3.*s1.^2.*s3.^2+ ...
  0.204800000000000000E5.*c1.^2.*c3.*s1.^2.*s3.^2+( ...
  -0.116811851851851852E5).*c3.^2.*s1.^2.*s3.^2+( ...
  -0.682666666666666667E4).*c1.*c3.^2.*s1.^2.*s3.^2+ ...
  0.227555555555555556E4.*c1.^2.*c3.^2.*s1.^2.*s3.^2+ ...
  0.230400000000000000E5.*s1.^4.*s3.^2+0.102400000000000000E5.*c3.* ...
  s1.^4.*s3.^2+0.113777777777777778E4.*c3.^2.*s1.^4.*s3.^2).^(-1),( ...
  0.E-37.*c1.*s3+0.E-37.*c1.^2.*s3+0.E-38.*c1.^2.*c3.*s3+0.E-38.* ...
  c1.*c3.^2.*s3+(-0.262826666666666667E6).*s1.*s3+ ...
  0.123618000000000000E6.*c1.*s1.*s3+0.576000000000000000E5.*c1.^2.* ...
  s1.*s3+0.658706666666666667E5.*c1.*c3.*s1.*s3+ ...
  0.256000000000000000E5.*c1.^2.*c3.*s1.*s3+( ...
  -0.292029629629629630E5).*c3.^2.*s1.*s3+0.853333333333333333E4.* ...
  c1.*c3.^2.*s1.*s3+0.284444444444444444E4.*c1.^2.*c3.^2.*s1.*s3+ ...
  0.E-37.*s1.^2.*s3+0.E-38.*c3.*s1.^2.*s3+0.576000000000000000E5.* ...
  s1.^3.*s3+0.256000000000000000E5.*c3.*s1.^3.*s3+ ...
  0.284444444444444444E4.*c3.^2.*s1.^3.*s3).*( ...
  0.175621873777777778E7+0.E-37.*c1+(-0.236544000000000000E6).* ...
  c1.^2+0.129863203555555556E7.*c3+0.315392000000000000E6.*c1.*c3+( ...
  -0.105130666666666667E6).*c1.^2.*c3+(-0.358315944691358025E6).* ...
  c3.^2+0.700871111111111111E5.*c1.*c3.^2+0.770228148148148148E5.* ...
  c1.^2.*c3.^2+(-0.440262272592592593E6).*c3.^3+( ...
  -0.118272000000000000E6).*c1.*c3.^3+0.394240000000000000E5.* ...
  c1.^2.*c3.^3+(-0.112599780740740741E6).*c3.^4+( ...
  -0.262826666666666667E5).*c1.*c3.^4+0.438044444444444444E4.* ...
  c1.^2.*c3.^4+(-0.175217777777777778E5).*c3.^5+0.E-39.*c1.*c3.^5+ ...
  0.E-39.*c3.^6+0.E-36.*s1+0.E-37.*c1.*s1+0.E-37.*c3.*s1+0.E-37.* ...
  c1.*c3.*s1+0.E-37.*c3.^2.*s1+0.E-37.*c1.*c3.^2.*s1+0.E-37.*c3.^3.* ...
  s1+0.E-38.*c1.*c3.^3.*s1+0.E-38.*c3.^4.*s1+0.E-39.*c1.*c3.^4.*s1+ ...
  0.E-39.*c3.^5.*s1+(-0.384885600000000000E6).*s1.^2+( ...
  -0.263220266666666667E6).*c3.*s1.^2+0.843654037037037037E5.* ...
  c3.^2.*s1.^2+0.941564888888888889E5.*c3.^3.*s1.^2+ ...
  0.224875111111111111E5.*c3.^4.*s1.^2+0.170666666666666667E4.* ...
  c3.^5.*s1.^2+(-0.171060266666666667E6).*c1.^2.*s3.^2+ ...
  0.230400000000000000E5.*c1.^4.*s3.^2+(-0.126490133333333333E6).* ...
  c1.^2.*c3.*s3.^2+(-0.307200000000000000E5).*c1.^3.*c3.*s3.^2+ ...
  0.102400000000000000E5.*c1.^4.*c3.*s3.^2+(-0.292466962962962963E5) ...
  .*c1.^2.*c3.^2.*s3.^2+(-0.682666666666666667E4).*c1.^3.*c3.^2.* ...
  s3.^2+0.113777777777777778E4.*c1.^4.*c3.^2.*s3.^2+( ...
  -0.455111111111111111E4).*c1.^2.*c3.^3.*s3.^2+0.E-37.*c1.*s1.* ...
  s3.^2+0.E-37.*c1.*c3.*s1.*s3.^2+0.E-38.*c1.*c3.^2.*s1.*s3.^2+( ...
  -0.105130666666666667E6).*s1.^2.*s3.^2+0.460800000000000000E5.* ...
  c1.^2.*s1.^2.*s3.^2+(-0.525653333333333333E5).*c3.*s1.^2.*s3.^2+( ...
  -0.307200000000000000E5).*c1.*c3.*s1.^2.*s3.^2+ ...
  0.204800000000000000E5.*c1.^2.*c3.*s1.^2.*s3.^2+( ...
  -0.116811851851851852E5).*c3.^2.*s1.^2.*s3.^2+( ...
  -0.682666666666666667E4).*c1.*c3.^2.*s1.^2.*s3.^2+ ...
  0.227555555555555556E4.*c1.^2.*c3.^2.*s1.^2.*s3.^2+ ...
  0.230400000000000000E5.*s1.^4.*s3.^2+0.102400000000000000E5.*c3.* ...
  s1.^4.*s3.^2+0.113777777777777778E4.*c3.^2.*s1.^4.*s3.^2).^(-1),(( ...
  -0.329291013333333333E6).*c3+0.E-37.*c1.*c3+ ...
  0.443520000000000000E5.*c1.^2.*c3+(-0.243493506666666667E6).* ...
  c3.^2+(-0.591360000000000000E5).*c1.*c3.^2+ ...
  0.197120000000000000E5.*c1.^2.*c3.^2+(-0.562998903703703704E5).* ...
  c3.^3+(-0.131413333333333333E5).*c1.*c3.^3+ ...
  0.219022222222222222E4.*c1.^2.*c3.^3+(-0.876088888888888889E4).* ...
  c3.^4+0.E-39.*c1.*c3.^4+0.E-39.*c3.^5+0.E-37.*c3.*s1+0.E-38.*c1.* ...
  c3.*s1+0.E-38.*c3.^2.*s1+0.E-38.*c1.*c3.^2.*s1+0.E-38.*c3.^3.*s1+ ...
  0.E-39.*c1.*c3.^3.*s1+0.E-39.*c3.^4.*s1+0.721660500000000000E5.* ...
  c3.*s1.^2+0.493538000000000000E5.*c3.^2.*s1.^2+ ...
  0.112437555555555556E5.*c3.^3.*s1.^2+0.853333333333333333E3.* ...
  c3.^4.*s1.^2).*(0.175621873777777778E7+0.E-37.*c1+( ...
  -0.236544000000000000E6).*c1.^2+0.129863203555555556E7.*c3+ ...
  0.315392000000000000E6.*c1.*c3+(-0.105130666666666667E6).*c1.^2.* ...
  c3+(-0.358315944691358025E6).*c3.^2+0.700871111111111111E5.*c1.* ...
  c3.^2+0.770228148148148148E5.*c1.^2.*c3.^2+( ...
  -0.440262272592592593E6).*c3.^3+(-0.118272000000000000E6).*c1.* ...
  c3.^3+0.394240000000000000E5.*c1.^2.*c3.^3+( ...
  -0.112599780740740741E6).*c3.^4+(-0.262826666666666667E5).*c1.* ...
  c3.^4+0.438044444444444444E4.*c1.^2.*c3.^4+( ...
  -0.175217777777777778E5).*c3.^5+0.E-39.*c1.*c3.^5+0.E-39.*c3.^6+ ...
  0.E-36.*s1+0.E-37.*c1.*s1+0.E-37.*c3.*s1+0.E-37.*c1.*c3.*s1+ ...
  0.E-37.*c3.^2.*s1+0.E-37.*c1.*c3.^2.*s1+0.E-37.*c3.^3.*s1+0.E-38.* ...
  c1.*c3.^3.*s1+0.E-38.*c3.^4.*s1+0.E-39.*c1.*c3.^4.*s1+0.E-39.* ...
  c3.^5.*s1+(-0.384885600000000000E6).*s1.^2+( ...
  -0.263220266666666667E6).*c3.*s1.^2+0.843654037037037037E5.* ...
  c3.^2.*s1.^2+0.941564888888888889E5.*c3.^3.*s1.^2+ ...
  0.224875111111111111E5.*c3.^4.*s1.^2+0.170666666666666667E4.* ...
  c3.^5.*s1.^2+(-0.171060266666666667E6).*c1.^2.*s3.^2+ ...
  0.230400000000000000E5.*c1.^4.*s3.^2+(-0.126490133333333333E6).* ...
  c1.^2.*c3.*s3.^2+(-0.307200000000000000E5).*c1.^3.*c3.*s3.^2+ ...
  0.102400000000000000E5.*c1.^4.*c3.*s3.^2+(-0.292466962962962963E5) ...
  .*c1.^2.*c3.^2.*s3.^2+(-0.682666666666666667E4).*c1.^3.*c3.^2.* ...
  s3.^2+0.113777777777777778E4.*c1.^4.*c3.^2.*s3.^2+( ...
  -0.455111111111111111E4).*c1.^2.*c3.^3.*s3.^2+0.E-37.*c1.*s1.* ...
  s3.^2+0.E-37.*c1.*c3.*s1.*s3.^2+0.E-38.*c1.*c3.^2.*s1.*s3.^2+( ...
  -0.105130666666666667E6).*s1.^2.*s3.^2+0.460800000000000000E5.* ...
  c1.^2.*s1.^2.*s3.^2+(-0.525653333333333333E5).*c3.*s1.^2.*s3.^2+( ...
  -0.307200000000000000E5).*c1.*c3.*s1.^2.*s3.^2+ ...
  0.204800000000000000E5.*c1.^2.*c3.*s1.^2.*s3.^2+( ...
  -0.116811851851851852E5).*c3.^2.*s1.^2.*s3.^2+( ...
  -0.682666666666666667E4).*c1.*c3.^2.*s1.^2.*s3.^2+ ...
  0.227555555555555556E4.*c1.^2.*c3.^2.*s1.^2.*s3.^2+ ...
  0.230400000000000000E5.*s1.^4.*s3.^2+0.102400000000000000E5.*c3.* ...
  s1.^4.*s3.^2+0.113777777777777778E4.*c3.^2.*s1.^4.*s3.^2).^(-1),( ...
  0.658582026666666667E7+0.E-36.*c1+(-0.887040000000000000E6).* ...
  c1.^2+0.486987013333333333E7.*c3+0.118272000000000000E7.*c1.*c3+( ...
  -0.394240000000000000E6).*c1.^2.*c3+0.112599780740740741E7.*c3.^2+ ...
  0.262826666666666667E6.*c1.*c3.^2+(-0.438044444444444444E5).* ...
  c1.^2.*c3.^2+0.175217777777777778E6.*c3.^3+0.E-38.*c1.*c3.^3+ ...
  0.E-38.*c3.^4+0.E-36.*s1+0.E-36.*c1.*s1+0.E-36.*c3.*s1+0.E-37.* ...
  c1.*c3.*s1+0.E-37.*c3.^2.*s1+0.E-38.*c1.*c3.^2.*s1+0.E-38.*c3.^3.* ...
  s1+(-0.144332100000000000E7).*s1.^2+(-0.987076000000000000E6).* ...
  c3.*s1.^2+(-0.224875111111111111E6).*c3.^2.*s1.^2+( ...
  -0.170666666666666667E5).*c3.^3.*s1.^2).*(0.175621873777777778E7+ ...
  0.E-37.*c1+(-0.236544000000000000E6).*c1.^2+ ...
  0.129863203555555556E7.*c3+0.315392000000000000E6.*c1.*c3+( ...
  -0.105130666666666667E6).*c1.^2.*c3+(-0.358315944691358025E6).* ...
  c3.^2+0.700871111111111111E5.*c1.*c3.^2+0.770228148148148148E5.* ...
  c1.^2.*c3.^2+(-0.440262272592592593E6).*c3.^3+( ...
  -0.118272000000000000E6).*c1.*c3.^3+0.394240000000000000E5.* ...
  c1.^2.*c3.^3+(-0.112599780740740741E6).*c3.^4+( ...
  -0.262826666666666667E5).*c1.*c3.^4+0.438044444444444444E4.* ...
  c1.^2.*c3.^4+(-0.175217777777777778E5).*c3.^5+0.E-39.*c1.*c3.^5+ ...
  0.E-39.*c3.^6+0.E-36.*s1+0.E-37.*c1.*s1+0.E-37.*c3.*s1+0.E-37.* ...
  c1.*c3.*s1+0.E-37.*c3.^2.*s1+0.E-37.*c1.*c3.^2.*s1+0.E-37.*c3.^3.* ...
  s1+0.E-38.*c1.*c3.^3.*s1+0.E-38.*c3.^4.*s1+0.E-39.*c1.*c3.^4.*s1+ ...
  0.E-39.*c3.^5.*s1+(-0.384885600000000000E6).*s1.^2+( ...
  -0.263220266666666667E6).*c3.*s1.^2+0.843654037037037037E5.* ...
  c3.^2.*s1.^2+0.941564888888888889E5.*c3.^3.*s1.^2+ ...
  0.224875111111111111E5.*c3.^4.*s1.^2+0.170666666666666667E4.* ...
  c3.^5.*s1.^2+(-0.171060266666666667E6).*c1.^2.*s3.^2+ ...
  0.230400000000000000E5.*c1.^4.*s3.^2+(-0.126490133333333333E6).* ...
  c1.^2.*c3.*s3.^2+(-0.307200000000000000E5).*c1.^3.*c3.*s3.^2+ ...
  0.102400000000000000E5.*c1.^4.*c3.*s3.^2+(-0.292466962962962963E5) ...
  .*c1.^2.*c3.^2.*s3.^2+(-0.682666666666666667E4).*c1.^3.*c3.^2.* ...
  s3.^2+0.113777777777777778E4.*c1.^4.*c3.^2.*s3.^2+( ...
  -0.455111111111111111E4).*c1.^2.*c3.^3.*s3.^2+0.E-37.*c1.*s1.* ...
  s3.^2+0.E-37.*c1.*c3.*s1.*s3.^2+0.E-38.*c1.*c3.^2.*s1.*s3.^2+( ...
  -0.105130666666666667E6).*s1.^2.*s3.^2+0.460800000000000000E5.* ...
  c1.^2.*s1.^2.*s3.^2+(-0.525653333333333333E5).*c3.*s1.^2.*s3.^2+( ...
  -0.307200000000000000E5).*c1.*c3.*s1.^2.*s3.^2+ ...
  0.204800000000000000E5.*c1.^2.*c3.*s1.^2.*s3.^2+( ...
  -0.116811851851851852E5).*c3.^2.*s1.^2.*s3.^2+( ...
  -0.682666666666666667E4).*c1.*c3.^2.*s1.^2.*s3.^2+ ...
  0.227555555555555556E4.*c1.^2.*c3.^2.*s1.^2.*s3.^2+ ...
  0.230400000000000000E5.*s1.^4.*s3.^2+0.102400000000000000E5.*c3.* ...
  s1.^4.*s3.^2+0.113777777777777778E4.*c3.^2.*s1.^4.*s3.^2).^(-1)]; 

C=[(-10/3).*c1.*(9+2.*c3).*qp(6)+(20/3).*qp(8).*s1.*s3+(100/9).*(qp(6).*(( ...
  -9/5).*s1+(-2/5).*c3.*s1)+(-1).*qp(8).*((3/5).*s3+(2/5).*c1.*s3+( ...
  4/15).*c3.*s3)),(20/3).*(8+c1.*(9+2.*c3)).*qp(3)+(10/3).*c1.*(9+2.* ...
  c3).*qp(6)+(-20/3).*qp(8).*s1.*s3+(-100/9).*(qp(6).*((-9/5).*s1+(-2/5).* ...
  c3.*s1)+(-1).*qp(8).*((3/5).*s3+(2/5).*c1.*s3+(4/15).*c3.*s3)),(-1) ...
  .*c1.*(9+2.*c3).*(qp(3)+qp(6))+2.*qp(8).*s1.*s3+(10/3).*((qp(3)+qp(6)).*(( ...
  -9/5).*s1+(-2/5).*c3.*s1)+(-1).*qp(8).*((2/5).*c1.*s3+(4/15).*c3.* ...
  s3)),0,(-2).*c1.*c3.*qp(8)+2.*(qp(3)+qp(6)).*s1.*s3+(10/3).*((-2/5).* ...
  c3.*qp(8).*s1+(-1).*qp(6).*((2/5).*c1.*s3+(4/15).*c3.*s3)+(-1).*qp(3).*( ...
  (3/5).*s3+(2/5).*c1.*s3+(4/15).*c3.*s3));(-20/3).*(8+c1.*(9+2.*c3) ...
  ).*qp(3)+(-10/3).*c1.*(9+2.*c3).*qp(6)+(20/3).*qp(8).*s1.*s3+(-100/9).*( ...
  qp(6).*((-9/5).*s1+(-2/5).*c3.*s1)+(-1).*qp(8).*((3/5).*s3+(2/5).*c1.* ...
  s3+(4/15).*c3.*s3)),(10/3).*c1.*(9+2.*c3).*qp(6)+(-20/3).*qp(8).*s1.* ...
  s3+(100/9).*(qp(6).*((-9/5).*s1+(-2/5).*c3.*s1)+(-1).*qp(8).*((3/5).* ...
  s3+(2/5).*c1.*s3+(4/15).*c3.*s3)),(-1).*c1.*(9+2.*c3).*(qp(3)+qp(6))+ ...
  2.*qp(8).*s1.*s3+(-10/3).*((qp(3)+qp(6)).*((-9/5).*s1+(-2/5).*c3.*s1)+( ...
  -1).*qp(8).*((2/5).*c1.*s3+(4/15).*c3.*s3)),0,(-2).*c1.*c3.*qp(8)+2.*( ...
  qp(3)+qp(6)).*s1.*s3+(-10/3).*((-2/5).*c3.*qp(8).*s1+(-1).*qp(6).*((2/5).* ...
  c1.*s3+(4/15).*c3.*s3)+(-1).*qp(3).*((3/5).*s3+(2/5).*c1.*s3+(4/15) ...
  .*c3.*s3));(10/3).*(qp(3).*((9/5).*s1+(2/5).*c3.*s1)+(-4/75).*c3.* ...
  qp(8).*s3),(-10/3).*(qp(3).*((9/5).*s1+(2/5).*c3.*s1)+(-4/75).*c3.* ...
  qp(8).*s3),qp(8).*((-3/5).*s3+(-4/15).*c3.*s3),0,(-4/15).*c3.*qp(3).*s3+ ...
  qp(6).*((-3/5).*s3+(-4/15).*c3.*s3);0,0,0,0,(-2).*qp(8).*s3;(10/3).*(( ...
  4/75).*c3.*qp(6).*s3+qp(3).*((3/5).*s3+(2/5).*c1.*s3+(4/15).*c3.*s3)), ...
  (-10/3).*((4/75).*c3.*qp(6).*s3+qp(3).*((3/5).*s3+(2/5).*c1.*s3+(4/15) ...
  .*c3.*s3)),(4/15).*c3.*qp(3).*s3+(-1).*qp(6).*((-3/5).*s3+(-4/15).* ...
  c3.*s3),0,0];
D=[0;0;0;0.392400000000000000E3;0.196200000000000000E2.*c3];
B=[0.266666666666666667E2,0,0,0,0;
    0,0.266666666666666667E2,0,0,0;
    0,0,1,0,0;0,0,0,1,0;0,0,0,0,1];



zp=invQ*(B*u-C*z-D);
